simulink model "TSR_Scenario_001_cs"  (R2014b)
settings: Solver=ode5  SolverMode=SingleTasking  StartTime=0.0  StopTime=inf  FixedStep=1/100  RelTol=1e-3
PreLoadFcn:
  | mbxruntime.callbacks.PreLoadFcn(bdroot);
  | check_NUTS_defined;
  | 
  | assignin('base',['model_closed_' bdroot],false);
  | 
  | addpath('../includes_TSR/includes_TSR');
  | 
  | switch version('-release')
  | case {'2010a', '2010b', '2011a'}
  | addpath('../includes_TSR/ML2010b');
  | otherwise
  | addpath('../includes_TSR/ML2011b');
  | end
PostLoadFcn:
  | mbxruntime.callbacks.PostLoadFcn(bdroot);
InitFcn:
  | mbxruntime.callbacks.InitFcn(bdroot);
StartFcn:
  | mbxruntime.callbacks.StartFcn(bdroot);
StopFcn:
  | mbxruntime.callbacks.StopFcn(bdroot);
model workspace: external: MAT-File .\TSR_Scenario_001_cs_hws.mat (data not in the file)
undefined symbols (not defined in the file or in its folder): InitImageOutputDir, mbxruntime, OrientationPitch, OrientationRoll, PositionX, PositionY, PositionZ, tabledata, warningInitialVelocity, x0
undefined symbols (not defined in the file): SteeringColumn, SteeringWheel, TSR_Scenario_001_cs_0469e6db089af631, TSR_Scenario_001_cs_0511100212e7bc8e, TSR_Scenario_001_cs_0e7e9ae969427aac, TSR_Scenario_001_cs_1093386e49c2fe1f, TSR_Scenario_001_cs_112063adae8cf595, TSR_Scenario_001_cs_20f00d93cd5331c2, TSR_Scenario_001_cs_23e3512474fbfadc, TSR_Scenario_001_cs_366523e1554c6bf4, TSR_Scenario_001_cs_37bce4982c67337a, TSR_Scenario_001_cs_44e6164a5df50f45, TSR_Scenario_001_cs_4963ce12e7ff3247, TSR_Scenario_001_cs_4b3e01fa729ce73a, TSR_Scenario_001_cs_519c34727ce9f069, TSR_Scenario_001_cs_5b66ab60038399a1, TSR_Scenario_001_cs_5baa165dfa1afdcb, TSR_Scenario_001_cs_5f993ce39fa6372c, TSR_Scenario_001_cs_613fdf28e3ff7437, TSR_Scenario_001_cs_67b1406af835d622, TSR_Scenario_001_cs_6ad990c290286b94, TSR_Scenario_001_cs_6c412b69295984e1, TSR_Scenario_001_cs_6d4c0c06b1585ef3, TSR_Scenario_001_cs_6dd019d071bf1235, TSR_Scenario_001_cs_6e9f5883f1a78533, TSR_Scenario_001_cs_80f7223d9ac35404, TSR_Scenario_001_cs_8562b82d3c89ae57, TSR_Scenario_001_cs_8a3a0181ab0babfe, TSR_Scenario_001_cs_8c997348ce80deaf, TSR_Scenario_001_cs_925bd6a073d9fe25, TSR_Scenario_001_cs_961436216add6114, TSR_Scenario_001_cs_991a7959256b2c84, TSR_Scenario_001_cs_9a95ce2c2e753616, TSR_Scenario_001_cs_a98aa9562e8552a9, TSR_Scenario_001_cs_ab44ae81dbfb58cd, TSR_Scenario_001_cs_Actros_2541_2_Path_pathUniqueID, TSR_Scenario_001_cs_ae74836ade6bff5a, TSR_Scenario_001_cs_Audi_A8_1_Dynamics_Simple_initialPitch, TSR_Scenario_001_cs_Audi_A8_1_Dynamics_Simple_initialRoll, TSR_Scenario_001_cs_Audi_A8_1_Dynamics_Simple_initialX, TSR_Scenario_001_cs_Audi_A8_1_Dynamics_Simple_initialY, TSR_Scenario_001_cs_Audi_A8_1_Dynamics_Simple_initialYaw, TSR_Scenario_001_cs_Audi_A8_1_Dynamics_Simple_initialZ, TSR_Scenario_001_cs_Audi_A8_2_Path_pathUniqueID, TSR_Scenario_001_cs_Audi_A8_2_SpeedProfile_speedProfileUniqueID, TSR_Scenario_001_cs_b2eca4eb2fce349a, TSR_Scenario_001_cs_b7bac209c1f2549f, TSR_Scenario_001_cs_bf3dccb66d3255a4, TSR_Scenario_001_cs_bf4c1a5315e3f716, TSR_Scenario_001_cs_BMW_Z3_1_Path_pathUniqueID, TSR_Scenario_001_cs_BMW_Z3_1_SpeedProfile_speedProfileUniqueID, TSR_Scenario_001_cs_BMW_Z3_2_Path_pathUniqueID, TSR_Scenario_001_cs_BMW_Z3_2_SpeedProfile_speedProfileUniqueID, TSR_Scenario_001_cs_c4c8fc4bdece03a9, TSR_Scenario_001_cs_c964c86aa54ad92e, TSR_Scenario_001_cs_cb64d1ef85329755, TSR_Scenario_001_cs_Citroen_C3_1_Path_pathUniqueID, TSR_Scenario_001_cs_Citroen_C3_2_Path_pathUniqueID, TSR_Scenario_001_cs_Citroen_C3_3_Path_pathUniqueID, TSR_Scenario_001_cs_Citroen_C3_4_Path_pathUniqueID ... (+25)
libraries: simulink x21, PreScanSimulinkLibrary x17, simulink_extras x13
(part 1 of 30)
CloseFcn:
  | mbxruntime.callbacks.CloseFcn(bdroot);
  | evalin('base',['clear model_closed_' bdroot]);
settings Model: Creator=PRESCAN  LastModifiedBy=jenkins
settings DataIOCC: SignalLoggingSaveFormat=ModelDataLogs
settings OptimizationCC: InlineParams=on  ExpressionDepthLimit=2147483647  InitFltsAndDblsToZero=on
settings DebuggingCC: SaveWithParameterizedLinksMsg=none  UnderspecifiedInitializationDetection=Classic  MergeDetectMultiDrivingBlocksExec=none  SignalResolutionControl=TryResolveAllWithWarning  SolverPrmCheckMsg=none  MultiTaskDSMMsg=warning  MultiTaskCondExecSysMsg=none  FcnCallInpInsideContextMsg=UseLocalSettings  StateNameClashWarn=warning
settings ModelReferenceCC: UpdateModelReferenceTargets=IfOutOfDate
settings SFSimCC: SimParseCustomCode=off
settings SFSimCC: SimCustomHeaderCode=|
  | #include "prescan.h"
  | #include "prescan_platform.h"
settings RTWCC: IncludeERTFirstTime=on
settings GRTTargetCC: TargetFcnLib=ansi_tfl_tmw.mat  CombineOutputUpdateFcns=off  GRTInterface=on

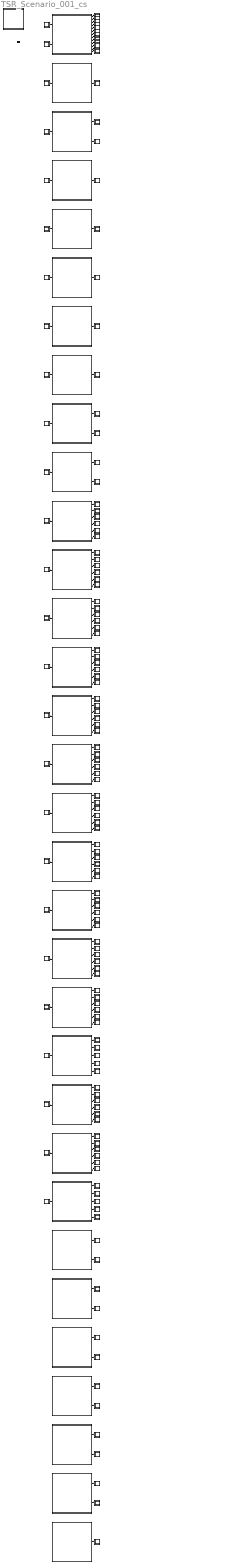
== system TSR_Scenario_001_cs ==
  note: Regenerate
  note: Simulink Mode
  note: Open Useful Blocks
  note: 2020.1.0
  note: Version:
  note: Author(s):
  note: N.A.
  note: Descriptive text:
  note: Demo Help
  note: ======
      | Num ID
      | ======
      | 1
      | 483
      | 484
      | 485
      | 828
      | 830
      | 486
      | 838
      | 959
      | 992
      | 999
      | 1001
      | 1002
      | 1003
      | 1004
      | 1005
      | 1006
      | 1007
      | 1008
      | 1009
      | 1010
      | 1011
      | 1012
      | 1000
  note: =============
      | OBU-Beacon ID
      | =============
  note: =======
      | Type ID
      | =======
      | 1
      | 3
      | 3
      | 7
      | 3
      | 7
      | 3
      | 1
      | 1
      | 1
      | 1
      | 1
      | 1
      | 1
      | 1
      | 1
      | 1
      | 1
      | 1
      | 1
      | 1
      | 1
      | 1
      | 3
  note: ========
      | Type Tag
      | ========
      | Car
      | Truck\Bus
      | Truck\Bus
      | Trailer
      | Truck\Bus
      | Trailer
      | Truck\Bus
      | Car
      | Car
      | Car
      | Car
      | Car
      | Car
      | Car
      | Car
      | Car
      | Car
      | Car
      | Car
      | Car
      | Car
      | Car
      | Car
      | Truck\Bus
  note: ==
      | SD
      | ==
      | Y
      | Y
      | Y
      | Y
      | Y
      | Y
      | Y
      | Y
      | Y
      | Y
      | Y
      | Y
      | Y
      | Y
      | Y
      | Y
      | Y
      | Y
      | Y
      | Y
      | Y
      | Y
      | Y
      | Y
  note: ==
      | CD
      | ==
      | N
      | N
      | N
      | N
      | N
      | N
      | N
      | N
      | N
      | N
      | N
      | N
      | N
      | N
      | N
      | N
      | N
      | N
      | N
      | N
      | N
      | N
      | N
      | N
  note: =======================
      | Name
      | =======================
      | Audi_A8_1
      | Nissan_Cabstar_1
      | Actros_1860_1
      | ContainerTrailer_DoubleAxle_1
      | Actros_1860_2
      | ContainerTrailer_DoubleAxle_2
      | Actros_2541_1
      | Toyota_Previa_1
      | Mazda_RX8_1
      | Mazda_RX8_2
      | Ford_Fiesta_1
      | BMW_Z3_1
      | Audi_A8_2
      | Citroen_C3_1
      | Citroen_C3_2
      | Toyota_Yaris_1
      | Fiat_Bravo_1
      | Citroen_C3_3
      | Toyota_Previa_2
      | Mazda_RX8_3
      | Fiat_Bravo_2
      | BMW_Z3_2
      | Citroen_C3_4
      | Actros_2541_2
  Actros_1860_1 : Subsystem  Tag=WorldObjectSubSystem  InitFcn=UniqueId = '1580';
      mask init:
      | modelPath = GenericModelHelper.getGenericModelFilePath('ModelDepo','Vehicles\Mercedes_Actros_1860\Mercedes_Actros_1860.pgmb','f4d262a59d21672e46677209b578f5e0');imagePath = GenericModelHelper.getCompilationPicture(modelPath, 'Mercedes_Actros_1860_HighPoly.png');
      mask Display: image(imread(imagePath));color('white');text(0, 0, ' ID=484\n')
  Actros_1860_2 : Subsystem  Tag=WorldObjectSubSystem  InitFcn=UniqueId = '1584';
      mask init: same as TSR_Scenario_001_cs/Actros_1860_1
      mask Display: image(imread(imagePath));color('white');text(0, 0, ' ID=828\n')
  Actros_2541_1 : Subsystem  Tag=WorldObjectSubSystem  InitFcn=UniqueId = '1588';
      mask init:
      | modelPath = GenericModelHelper.getGenericModelFilePath('ModelDepo','Vehicles\Mercedes_Actros_2541\Mercedes_Actros_2541.pgmb','2272788c542945e1b586df6742792b5a');imagePath = GenericModelHelper.getCompilationPicture(modelPath, 'Mercedes_Actros_2541_HighPoly.png');
      mask Display: image(imread(imagePath));color('white');text(0, 0, ' ID=486\n')
  Actros_2541_2 : Subsystem  Tag=WorldObjectSubSystem  InitFcn=UniqueId = '2575';
      mask init: same as TSR_Scenario_001_cs/Actros_2541_1
      mask Display: image(imread(imagePath));color('white');text(0, 0, ' ID=1000\n')
  Audi_A8_1 : Subsystem  Tag=WorldObjectSubSystem  InitFcn=UniqueId = '253';
      mask init:
      | modelPath = GenericModelHelper.getGenericModelFilePath('ModelDepo','Vehicles\Audi_A8\Audi_A8.pgmb','e33fe1ddcf3e8ae97caccbc8f2fa74ac');imagePath = GenericModelHelper.getCompilationPicture(modelPath, 'Audi_A8_HighPoly.png');
      mask Display: image(imread(imagePath));color('white');text(0, 0, ' ID=1\n')
  Audi_A8_1_Brake_light_left : Subsystem  Tag=actuator/BrakeLightL  Priority=0  LoadFcn=load('PreScanVisuLightActuatorData');load('PrescanRPYData');load('PrescanXYZData');load('PreScanRGBData')  mask(PreScan Sink Block: VisuActiveLight){}
      mask help:
      | The VisuActiveLight block provides a way for detailed animation of Light Sources, such as the indicator, brake, fog and main lights of a vehicle, or a light post.
      |
      | For more information, please click Help.
      settings: OpenFcn=open_system([gcb '/Actuator'],'mask')
      mask Help: eval('openHelp(209)')
      mask Display: image(imread('HeadLight.png'))
  Audi_A8_1_Brake_light_right : Subsystem  Tag=actuator/BrakeLightR  Priority=0  LoadFcn=load('PreScanVisuLightActuatorData');load('PrescanRPYData');load('PrescanXYZData');load('PreScanRGBData')  mask(PreScan Sink Block: VisuActiveLight){}
      mask help:
      | The VisuActiveLight block provides a way for detailed animation of Light Sources, such as the indicator, brake, fog and main lights of a vehicle, or a light post.
      |
      | For more information, please click Help.
      settings: OpenFcn=open_system([gcb '/Actuator'],'mask')
      mask Help: eval('openHelp(209)')
      mask Display: image(imread('HeadLight.png'))
  Audi_A8_1_Indicator_front_left : Subsystem  Tag=actuator/IndicatorFL  Priority=0  LoadFcn=load('PreScanVisuLightActuatorData');load('PrescanRPYData');load('PrescanXYZData');load('PreScanRGBData')  mask(PreScan Sink Block: VisuActiveLight){}
      mask help:
      | The VisuActiveLight block provides a way for detailed animation of Light Sources, such as the indicator, brake, fog and main lights of a vehicle, or a light post.
      |
      | For more information, please click Help.
      settings: OpenFcn=open_system([gcb '/Actuator'],'mask')
      mask Help: eval('openHelp(209)')
      mask Display: image(imread('HeadLight.png'))
  Audi_A8_1_Indicator_front_right : Subsystem  Tag=actuator/IndicatorFR  Priority=0  LoadFcn=load('PreScanVisuLightActuatorData');load('PrescanRPYData');load('PrescanXYZData');load('PreScanRGBData')  mask(PreScan Sink Block: VisuActiveLight){}
      mask help:
      | The VisuActiveLight block provides a way for detailed animation of Light Sources, such as the indicator, brake, fog and main lights of a vehicle, or a light post.
      |
      | For more information, please click Help.
      settings: OpenFcn=open_system([gcb '/Actuator'],'mask')
      mask Help: eval('openHelp(209)')
      mask Display: image(imread('HeadLight.png'))
  Audi_A8_1_Indicator_rear_left : Subsystem  Tag=actuator/IndicatorRL  Priority=0  LoadFcn=load('PreScanVisuLightActuatorData');load('PrescanRPYData');load('PrescanXYZData');load('PreScanRGBData')  mask(PreScan Sink Block: VisuActiveLight){}
      mask help:
      | The VisuActiveLight block provides a way for detailed animation of Light Sources, such as the indicator, brake, fog and main lights of a vehicle, or a light post.
      |
      | For more information, please click Help.
      settings: OpenFcn=open_system([gcb '/Actuator'],'mask')
      mask Help: eval('openHelp(209)')
      mask Display: image(imread('HeadLight.png'))
  Audi_A8_1_Indicator_rear_right : Subsystem  Tag=actuator/IndicatorRR  Priority=0  LoadFcn=load('PreScanVisuLightActuatorData');load('PrescanRPYData');load('PrescanXYZData');load('PreScanRGBData')  mask(PreScan Sink Block: VisuActiveLight){}
      mask help:
      | The VisuActiveLight block provides a way for detailed animation of Light Sources, such as the indicator, brake, fog and main lights of a vehicle, or a light post.
      |
      | For more information, please click Help.
      settings: OpenFcn=open_system([gcb '/Actuator'],'mask')
      mask Help: eval('openHelp(209)')
      mask Display: image(imread('HeadLight.png'))
  Audi_A8_2 : Subsystem  Tag=WorldObjectSubSystem  InitFcn=UniqueId = '1951';
      mask init: same as TSR_Scenario_001_cs/Audi_A8_1
      mask Display: image(imread(imagePath));color('white');text(0, 0, ' ID=1002\n')
  BMW_Z3_1 : Subsystem  Tag=WorldObjectSubSystem  InitFcn=UniqueId = '1948';
      mask init:
      | modelPath = GenericModelHelper.getGenericModelFilePath('ModelDepo','Vehicles\BMW_Z3\BMW_Z3.pgmb','9e6af5cc2d86218dad43975fd3a29d11');imagePath = GenericModelHelper.getCompilationPicture(modelPath, 'BMW_Z3_HighPoly.png');
      mask Display: image(imread(imagePath));color('white');text(0, 0, ' ID=1001\n')
  BMW_Z3_2 : Subsystem  Tag=WorldObjectSubSystem  InitFcn=UniqueId = '2024';
      mask init: same as TSR_Scenario_001_cs/BMW_Z3_1
      mask Display: image(imread(imagePath));color('white');text(0, 0, ' ID=1011\n')
  CameraSensor_1 : Subsystem  Tag=sensor/Camera/CameraSensor  Priority=30  mask(PreScan Source Block: Camera Sensor){}
      mask help: The Camera Sensor provides a color or monochrome image.
      settings: OpenFcn=open_system([gcb '/Sensor'],'mask')
      mask Help: eval('openHelp(457)')
      mask Display: image(imread('CameraSensor.png'))
  Citroen_C3_1 : Subsystem  Tag=WorldObjectSubSystem  InitFcn=UniqueId = '1955';
      mask init:
      | modelPath = GenericModelHelper.getGenericModelFilePath('ModelDepo','Vehicles\Citroen_C3\Citroen_C3.pgmb','e804ced06d50dbfc6a2202ab3ad01b0c');imagePath = GenericModelHelper.getCompilationPicture(modelPath, 'Citroen_C3_HighPoly.png');
      mask Display: image(imread(imagePath));color('white');text(0, 0, ' ID=1003\n')
  Citroen_C3_2 : Subsystem  Tag=WorldObjectSubSystem  InitFcn=UniqueId = '1958';
      mask init: same as TSR_Scenario_001_cs/Citroen_C3_1
      mask Display: image(imread(imagePath));color('white');text(0, 0, ' ID=1004\n')
  Citroen_C3_3 : Subsystem  Tag=WorldObjectSubSystem  InitFcn=UniqueId = '1967';
      mask init: same as TSR_Scenario_001_cs/Citroen_C3_1
      mask Display: image(imread(imagePath));color('white');text(0, 0, ' ID=1007\n')
  Citroen_C3_4 : Subsystem  Tag=WorldObjectSubSystem  InitFcn=UniqueId = '2027';
      mask init: same as TSR_Scenario_001_cs/Citroen_C3_1
      mask Display: image(imread(imagePath));color('white');text(0, 0, ' ID=1012\n')
  ContainerTrailer_DoubleAxle_1 : Subsystem  Tag=WorldObjectSubSystem  InitFcn=UniqueId = '1582';
      mask init:
      | modelPath = GenericModelHelper.getGenericModelFilePath('ModelDepo','Vehicles\Container\Container.pgmb','6d816eb34d08248d7edc89a1bf7f028c');imagePath = GenericModelHelper.getCompilationPicture(modelPath, 'Container_HighPoly.png');
      mask Display: image(imread(imagePath));color('white');text(0, 0, ' ID=485\n')
  ContainerTrailer_DoubleAxle_2 : Subsystem  Tag=WorldObjectSubSystem  InitFcn=UniqueId = '1586';
      mask init: same as TSR_Scenario_001_cs/ContainerTrailer_DoubleAxle_1
      mask Display: image(imread(imagePath));color('white');text(0, 0, ' ID=830\n')
  Controller : Subsystem  Description=8A3CD2955739A82C886C20AE3E253D78460D53180EE2C1B14CC08DF75A70BE77  Priority=-1  LoadFcn=load PreScanControllerData  mask(PreScan Simulation Controller){prescanversion='2020.1.0', ModelReferencing=off, TimeStep=1/100, ControlMode=0, PreScanExecutionMode=on, ControllerCount=0, ControllerIndex=0, ControllerOptions=''}
      mask prompts: prescanversion "PreScan Version"; ModelReferencing "Use Model Referencing"; TimeStep "Upload Period [s]"; ControlMode "Control Mode"; PreScanExecutionMode "Execution Mode"; ControllerCount "Controller Count"; ControllerIndex "Controller Index"; ControllerOptions "Controller Options"
      mask help:
      | Please do not remove this block from the compilation sheet,
      | as it connects the model to the PreScan environment.
      mask init:
      | model = bdroot(gcb);
      | ExperimentFile = mbxruntime.findExperimentFile(model,true); %relative path
      | 
      | [d1, d2, d3, prescandata] = prescan_Settings();
      | ModelDepo = fullfile(prescandata,'ModelDepo'); 
      | 
      | RTmode = mbxruntime.getRTMode(model);
      | 
      | SimulationMode = get_param(bdroot,'SimulationMode');
      | if strcmp(SimulationMode, 'rapid-accelerator')
      |     SimulationMode = 'external';
      | end
      | TargetName = get_param(bdroot,'SystemTargetFile');
      settings: ModelCloseFcn=assignin('base',['model_closed_' bdroot],true);
      mask Help: eval('openHelp(812)')
      mask Display: image(imread('prescanlogo.ico'))
  Fiat_Bravo_1 : Subsystem  Tag=WorldObjectSubSystem  InitFcn=UniqueId = '1964';
      mask init:
      | modelPath = GenericModelHelper.getGenericModelFilePath('ModelDepo','Vehicles\Fiat_Bravo\Fiat_Bravo.pgmb','a97eb0ec4093646e5d079d2ab9a2eab7');imagePath = GenericModelHelper.getCompilationPicture(modelPath, 'Fiat_Bravo_HighPoly.png');
      mask Display: image(imread(imagePath));color('white');text(0, 0, ' ID=1006\n')
  Fiat_Bravo_2 : Subsystem  Tag=WorldObjectSubSystem  InitFcn=UniqueId = '2021';
      mask init: same as TSR_Scenario_001_cs/Fiat_Bravo_1
      mask Display: image(imread(imagePath));color('white');text(0, 0, ' ID=1010\n')
  Ford_Fiesta_1 : Subsystem  Tag=WorldObjectSubSystem  InitFcn=UniqueId = '1934';
      mask init:
      | modelPath = GenericModelHelper.getGenericModelFilePath('ModelDepo','Vehicles\Ford_Fiesta\Ford_Fiesta.pgmb','fe2c7a73e0a60cba76689b71cd1bb76a');imagePath = GenericModelHelper.getCompilationPicture(modelPath, 'Ford_Fiesta_HighPoly.png');
      mask Display: image(imread(imagePath));color('white');text(0, 0, ' ID=999\n')
  HighwayOverhang_1 : Subsystem  Tag=WorldObjectSubSystem  InitFcn=UniqueId = '1876';
      mask init:
      | imagePath=which('HighwayOverhang.jpg');
      mask Display: image(imread(imagePath));color('white');text(0, 0, ' ID=115\n')
  HighwayOverhang_2 : Subsystem  Tag=WorldObjectSubSystem  InitFcn=UniqueId = '1877';
      mask init:
      | imagePath=which('HighwayOverhang.jpg');
      mask Display: image(imread(imagePath));color('white');text(0, 0, ' ID=973\n')
  HighwayOverhang_3 : Subsystem  Tag=WorldObjectSubSystem  InitFcn=UniqueId = '1890';
      mask init:
      | imagePath=which('HighwayOverhang.jpg');
      mask Display: image(imread(imagePath));color('white');text(0, 0, ' ID=985\n')
  HighwayOverhang_4 : Subsystem  Tag=WorldObjectSubSystem  InitFcn=UniqueId = '1898';
      mask init:
      | imagePath=which('HighwayOverhang.jpg');
      mask Display: image(imread(imagePath));color('white');text(0, 0, ' ID=988\n')
  HighwayOverhang_5 : Subsystem  Tag=WorldObjectSubSystem  InitFcn=UniqueId = '1909';
      mask init:
      | imagePath=which('HighwayOverhang.jpg');
      mask Display: image(imread(imagePath));color('white');text(0, 0, ' ID=993\n')
  HighwayOverhang_6 : Subsystem  Tag=WorldObjectSubSystem  InitFcn=UniqueId = '1914';
      mask init:
      | imagePath=which('HighwayOverhang.jpg');
      mask Display: image(imread(imagePath));color('white');text(0, 0, ' ID=994\n')
  HighwayOverhang_7 : Subsystem  Tag=WorldObjectSubSystem  InitFcn=UniqueId = '2612';
      mask init:
      | imagePath=which('HighwayOverhang.jpg');
      mask Display: image(imread(imagePath));color('white');text(0, 0, ' ID=1505\n')
  Mazda_RX8_1 : Subsystem  Tag=WorldObjectSubSystem  InitFcn=UniqueId = '1863';
      mask init:
      | modelPath = GenericModelHelper.getGenericModelFilePath('ModelDepo','Vehicles\Mazda_RX8\Mazda_RX8.pgmb','1e55a2e40efa576b7f4fb93bae35d605');imagePath = GenericModelHelper.getCompilationPicture(modelPath, 'Mazda_RX8_HighPoly.png');
      mask Display: image(imread(imagePath));color('white');text(0, 0, ' ID=959\n')
  Mazda_RX8_2 : Subsystem  Tag=WorldObjectSubSystem  InitFcn=UniqueId = '1929';
      mask init: same as TSR_Scenario_001_cs/Mazda_RX8_1
      mask Display: image(imread(imagePath));color('white');text(0, 0, ' ID=992\n')
  Mazda_RX8_3 : Subsystem  Tag=WorldObjectSubSystem  InitFcn=UniqueId = '1973';
      mask init: same as TSR_Scenario_001_cs/Mazda_RX8_1
      mask Display: image(imread(imagePath));color('white');text(0, 0, ' ID=1009\n')
  Nissan_Cabstar_1 : Subsystem  Tag=WorldObjectSubSystem  InitFcn=UniqueId = '1579';
      mask init:
      | modelPath = GenericModelHelper.getGenericModelFilePath('ModelDepo','Vehicles\Nissan_Cabstar\Nissan_Cabstar.pgmb','dd076fdae311093c5436e82e6c23dc23');imagePath = GenericModelHelper.getCompilationPicture(modelPath, 'Nissan_Cabstar_HighPoly.png');
      mask Display: image(imread(imagePath));color('white');text(0, 0, ' ID=483\n')
  PreScanTerminator : Subsystem  Tag=PreScanTerminator  Priority=999  LoadFcn=load PrescanTerminatorData  mask(PreScan Simulation Terminator){TimeStep=1/100}
      mask prompts: TimeStep "Upload Period [s]"
      mask help:
      | Please do not remove this block from the compilation sheet as it
      | connects the model to the PreScan environment.
      mask Help: eval('openHelp(812)')
      mask Display: image(imread('prescanlogo.ico'))
  SELF_Actros_1860_1 : Subsystem  Tag=sensor/SelfPort  Priority=30  LoadFcn=load('PreScanSelfSensorData.mat')  mask(PreScan Source Block: SELF){}
      mask help:
      | The SELF port shows (state) information of the actor itself. The outputs are position in the experiment's axis system and the GPS coordinates, and the object's absolute velocity and compass heading.
      |
      | For more information, please click Help.
      settings: OpenFcn=open_system([gcb '/Sensor'],'mask')
      mask Help: eval('openHelp(462)')
      mask Display: image(imread('GPS.png'))
  SELF_Actros_1860_2 : Subsystem  Tag=sensor/SelfPort  Priority=30  LoadFcn=load('PreScanSelfSensorData.mat')  mask(PreScan Source Block: SELF){}
      mask help:
      | The SELF port shows (state) information of the actor itself. The outputs are position in the experiment's axis system and the GPS coordinates, and the object's absolute velocity and compass heading.
      |
      | For more information, please click Help.
      settings: OpenFcn=open_system([gcb '/Sensor'],'mask')
      mask Help: eval('openHelp(462)')
      mask Display: image(imread('GPS.png'))
  SELF_Actros_2541_1 : Subsystem  Tag=sensor/SelfPort  Priority=30  LoadFcn=load('PreScanSelfSensorData.mat')  mask(PreScan Source Block: SELF){}
      mask help:
      | The SELF port shows (state) information of the actor itself. The outputs are position in the experiment's axis system and the GPS coordinates, and the object's absolute velocity and compass heading.
      |
      | For more information, please click Help.
      settings: OpenFcn=open_system([gcb '/Sensor'],'mask')
      mask Help: eval('openHelp(462)')
      mask Display: image(imread('GPS.png'))
  SELF_Actros_2541_2 : Subsystem  Tag=sensor/SelfPort  Priority=30  LoadFcn=load('PreScanSelfSensorData.mat')  mask(PreScan Source Block: SELF){}
      mask help:
      | The SELF port shows (state) information of the actor itself. The outputs are position in the experiment's axis system and the GPS coordinates, and the object's absolute velocity and compass heading.
      |
      | For more information, please click Help.
      settings: OpenFcn=open_system([gcb '/Sensor'],'mask')
      mask Help: eval('openHelp(462)')
      mask Display: image(imread('GPS.png'))
  SELF_Audi_A8_1 : Subsystem  Tag=sensor/SelfPort  Priority=30  LoadFcn=load('PreScanSelfSensorData.mat')  mask(PreScan Source Block: SELF){}
      mask help:
      | The SELF port shows (state) information of the actor itself. The outputs are position in the experiment's axis system and the GPS coordinates, and the object's absolute velocity and compass heading.
      |
      | For more information, please click Help.
      settings: OpenFcn=open_system([gcb '/Sensor'],'mask')
      mask Help: eval('openHelp(462)')
      mask Display: image(imread('GPS.png'))
  SELF_Audi_A8_2 : Subsystem  Tag=sensor/SelfPort  Priority=30  LoadFcn=load('PreScanSelfSensorData.mat')  mask(PreScan Source Block: SELF){}
      mask help:
      | The SELF port shows (state) information of the actor itself. The outputs are position in the experiment's axis system and the GPS coordinates, and the object's absolute velocity and compass heading.
      |
      | For more information, please click Help.
      settings: OpenFcn=open_system([gcb '/Sensor'],'mask')
      mask Help: eval('openHelp(462)')
      mask Display: image(imread('GPS.png'))
  SELF_BMW_Z3_1 : Subsystem  Tag=sensor/SelfPort  Priority=30  LoadFcn=load('PreScanSelfSensorData.mat')  mask(PreScan Source Block: SELF){}
      mask help:
      | The SELF port shows (state) information of the actor itself. The outputs are position in the experiment's axis system and the GPS coordinates, and the object's absolute velocity and compass heading.
      |
      | For more information, please click Help.
      settings: OpenFcn=open_system([gcb '/Sensor'],'mask')
      mask Help: eval('openHelp(462)')
      mask Display: image(imread('GPS.png'))
  SELF_BMW_Z3_2 : Subsystem  Tag=sensor/SelfPort  Priority=30  LoadFcn=load('PreScanSelfSensorData.mat')  mask(PreScan Source Block: SELF){}
      mask help:
      | The SELF port shows (state) information of the actor itself. The outputs are position in the experiment's axis system and the GPS coordinates, and the object's absolute velocity and compass heading.
      |
      | For more information, please click Help.
      settings: OpenFcn=open_system([gcb '/Sensor'],'mask')
      mask Help: eval('openHelp(462)')
      mask Display: image(imread('GPS.png'))
  SELF_Citroen_C3_1 : Subsystem  Tag=sensor/SelfPort  Priority=30  LoadFcn=load('PreScanSelfSensorData.mat')  mask(PreScan Source Block: SELF){}
      mask help:
      | The SELF port shows (state) information of the actor itself. The outputs are position in the experiment's axis system and the GPS coordinates, and the object's absolute velocity and compass heading.
      |
      | For more information, please click Help.
      settings: OpenFcn=open_system([gcb '/Sensor'],'mask')
      mask Help: eval('openHelp(462)')
      mask Display: image(imread('GPS.png'))
  SELF_Citroen_C3_2 : Subsystem  Tag=sensor/SelfPort  Priority=30  LoadFcn=load('PreScanSelfSensorData.mat')  mask(PreScan Source Block: SELF){}
      mask help:
      | The SELF port shows (state) information of the actor itself. The outputs are position in the experiment's axis system and the GPS coordinates, and the object's absolute velocity and compass heading.
      |
      | For more information, please click Help.
      settings: OpenFcn=open_system([gcb '/Sensor'],'mask')
      mask Help: eval('openHelp(462)')
      mask Display: image(imread('GPS.png'))
  SELF_Citroen_C3_3 : Subsystem  Tag=sensor/SelfPort  Priority=30  LoadFcn=load('PreScanSelfSensorData.mat')  mask(PreScan Source Block: SELF){}
      mask help:
      | The SELF port shows (state) information of the actor itself. The outputs are position in the experiment's axis system and the GPS coordinates, and the object's absolute velocity and compass heading.
      |
      | For more information, please click Help.
      settings: OpenFcn=open_system([gcb '/Sensor'],'mask')
      mask Help: eval('openHelp(462)')
      mask Display: image(imread('GPS.png'))
  SELF_Citroen_C3_4 : Subsystem  Tag=sensor/SelfPort  Priority=30  LoadFcn=load('PreScanSelfSensorData.mat')  mask(PreScan Source Block: SELF){}
      mask help:
      | The SELF port shows (state) information of the actor itself. The outputs are position in the experiment's axis system and the GPS coordinates, and the object's absolute velocity and compass heading.
      |
      | For more information, please click Help.
      settings: OpenFcn=open_system([gcb '/Sensor'],'mask')
      mask Help: eval('openHelp(462)')
      mask Display: image(imread('GPS.png'))
  SELF_ContainerTrailer_DoubleAxle_1 : Subsystem  Tag=sensor/SelfPort  Priority=30  LoadFcn=load('PreScanSelfSensorData.mat')  mask(PreScan Source Block: SELF){}
      mask help:
      | The SELF port shows (state) information of the actor itself. The outputs are position in the experiment's axis system and the GPS coordinates, and the object's absolute velocity and compass heading.
      |
      | For more information, please click Help.
      settings: OpenFcn=open_system([gcb '/Sensor'],'mask')
      mask Help: eval('openHelp(462)')
      mask Display: image(imread('GPS.png'))
  SELF_ContainerTrailer_DoubleAxle_2 : Subsystem  Tag=sensor/SelfPort  Priority=30  LoadFcn=load('PreScanSelfSensorData.mat')  mask(PreScan Source Block: SELF){}
      mask help:
      | The SELF port shows (state) information of the actor itself. The outputs are position in the experiment's axis system and the GPS coordinates, and the object's absolute velocity and compass heading.
      |
      | For more information, please click Help.
      settings: OpenFcn=open_system([gcb '/Sensor'],'mask')
      mask Help: eval('openHelp(462)')
      mask Display: image(imread('GPS.png'))
  SELF_Fiat_Bravo_1 : Subsystem  Tag=sensor/SelfPort  Priority=30  LoadFcn=load('PreScanSelfSensorData.mat')  mask(PreScan Source Block: SELF){}
      mask help:
      | The SELF port shows (state) information of the actor itself. The outputs are position in the experiment's axis system and the GPS coordinates, and the object's absolute velocity and compass heading.
      |
      | For more information, please click Help.
      settings: OpenFcn=open_system([gcb '/Sensor'],'mask')
      mask Help: eval('openHelp(462)')
      mask Display: image(imread('GPS.png'))
  SELF_Fiat_Bravo_2 : Subsystem  Tag=sensor/SelfPort  Priority=30  LoadFcn=load('PreScanSelfSensorData.mat')  mask(PreScan Source Block: SELF){}
      mask help:
      | The SELF port shows (state) information of the actor itself. The outputs are position in the experiment's axis system and the GPS coordinates, and the object's absolute velocity and compass heading.
      |
      | For more information, please click Help.
      settings: OpenFcn=open_system([gcb '/Sensor'],'mask')
      mask Help: eval('openHelp(462)')
      mask Display: image(imread('GPS.png'))
  SELF_Ford_Fiesta_1 : Subsystem  Tag=sensor/SelfPort  Priority=30  LoadFcn=load('PreScanSelfSensorData.mat')  mask(PreScan Source Block: SELF){}
      mask help:
      | The SELF port shows (state) information of the actor itself. The outputs are position in the experiment's axis system and the GPS coordinates, and the object's absolute velocity and compass heading.
      |
      | For more information, please click Help.
      settings: OpenFcn=open_system([gcb '/Sensor'],'mask')
      mask Help: eval('openHelp(462)')
      mask Display: image(imread('GPS.png'))
  SELF_Mazda_RX8_1 : Subsystem  Tag=sensor/SelfPort  Priority=30  LoadFcn=load('PreScanSelfSensorData.mat')  mask(PreScan Source Block: SELF){}
      mask help:
      | The SELF port shows (state) information of the actor itself. The outputs are position in the experiment's axis system and the GPS coordinates, and the object's absolute velocity and compass heading.
      |
      | For more information, please click Help.
      settings: OpenFcn=open_system([gcb '/Sensor'],'mask')
      mask Help: eval('openHelp(462)')
      mask Display: image(imread('GPS.png'))
  SELF_Mazda_RX8_2 : Subsystem  Tag=sensor/SelfPort  Priority=30  LoadFcn=load('PreScanSelfSensorData.mat')  mask(PreScan Source Block: SELF){}
      mask help:
      | The SELF port shows (state) information of the actor itself. The outputs are position in the experiment's axis system and the GPS coordinates, and the object's absolute velocity and compass heading.
      |
      | For more information, please click Help.
      settings: OpenFcn=open_system([gcb '/Sensor'],'mask')
      mask Help: eval('openHelp(462)')
      mask Display: image(imread('GPS.png'))
  SELF_Mazda_RX8_3 : Subsystem  Tag=sensor/SelfPort  Priority=30  LoadFcn=load('PreScanSelfSensorData.mat')  mask(PreScan Source Block: SELF){}
      mask help:
      | The SELF port shows (state) information of the actor itself. The outputs are position in the experiment's axis system and the GPS coordinates, and the object's absolute velocity and compass heading.
      |
      | For more information, please click Help.
      settings: OpenFcn=open_system([gcb '/Sensor'],'mask')
      mask Help: eval('openHelp(462)')
      mask Display: image(imread('GPS.png'))
  SELF_Nissan_Cabstar_1 : Subsystem  Tag=sensor/SelfPort  Priority=30  LoadFcn=load('PreScanSelfSensorData.mat')  mask(PreScan Source Block: SELF){}
      mask help:
      | The SELF port shows (state) information of the actor itself. The outputs are position in the experiment's axis system and the GPS coordinates, and the object's absolute velocity and compass heading.
      |
      | For more information, please click Help.
      settings: OpenFcn=open_system([gcb '/Sensor'],'mask')
      mask Help: eval('openHelp(462)')
      mask Display: image(imread('GPS.png'))
  SELF_Sphere_1 : Subsystem  Tag=sensor/SelfPort  Priority=30  LoadFcn=load('PreScanSelfSensorData.mat')  mask(PreScan Source Block: SELF){}
      mask help:
      | The SELF port shows (state) information of the actor itself. The outputs are position in the experiment's axis system and the GPS coordinates, and the object's absolute velocity and compass heading.
      |
      | For more information, please click Help.
      settings: OpenFcn=open_system([gcb '/Sensor'],'mask')
      mask Help: eval('openHelp(462)')
      mask Display: image(imread('GPS.png'))
  SELF_Toyota_Previa_1 : Subsystem  Tag=sensor/SelfPort  Priority=30  LoadFcn=load('PreScanSelfSensorData.mat')  mask(PreScan Source Block: SELF){}
      mask help:
      | The SELF port shows (state) information of the actor itself. The outputs are position in the experiment's axis system and the GPS coordinates, and the object's absolute velocity and compass heading.
      |
      | For more information, please click Help.
      settings: OpenFcn=open_system([gcb '/Sensor'],'mask')
      mask Help: eval('openHelp(462)')
      mask Display: image(imread('GPS.png'))
  SELF_Toyota_Previa_2 : Subsystem  Tag=sensor/SelfPort  Priority=30  LoadFcn=load('PreScanSelfSensorData.mat')  mask(PreScan Source Block: SELF){}
      mask help:
      | The SELF port shows (state) information of the actor itself. The outputs are position in the experiment's axis system and the GPS coordinates, and the object's absolute velocity and compass heading.
      |
      | For more information, please click Help.
      settings: OpenFcn=open_system([gcb '/Sensor'],'mask')
      mask Help: eval('openHelp(462)')
      mask Display: image(imread('GPS.png'))
  SELF_Toyota_Yaris_1 : Subsystem  Tag=sensor/SelfPort  Priority=30  LoadFcn=load('PreScanSelfSensorData.mat')  mask(PreScan Source Block: SELF){}
      mask help:
      | The SELF port shows (state) information of the actor itself. The outputs are position in the experiment's axis system and the GPS coordinates, and the object's absolute velocity and compass heading.
      |
      | For more information, please click Help.
      settings: OpenFcn=open_system([gcb '/Sensor'],'mask')
      mask Help: eval('openHelp(462)')
      mask Display: image(imread('GPS.png'))
  STATE_Actros_1860_1_bus : Subsystem  Tag=actuator/StatePort  Priority=0  LoadFcn=load('PreScanStateActuatorData.mat')  mask(PreScan Sink Block: State){}
      mask help:
      | The Actor State contains a vector signal of size (9x1), containing the following signals:
      |
      | -  Position    	(x,y,z)             	[m]
      | -  Velocity    	(vx,vy,vz)         	[m/s]
      | -  Angles       	(Roll, Pitch, Yaw)	[rad]
      |
      | The Actor state is defined in the global axis system.
      | The state is superponed on the Initial position defined in the GUI.
      |
      | For more information, please click Help.
      settings: OpenFcn=open_system([gcb '/Actuator'],'mask')
      mask Help: eval('openHelp(222)')
      mask Display: image(imread('State.png'))
  STATE_Actros_1860_2_bus : Subsystem  Tag=actuator/StatePort  Priority=0  LoadFcn=load('PreScanStateActuatorData.mat')  mask(PreScan Sink Block: State){}
      mask help:
      | The Actor State contains a vector signal of size (9x1), containing the following signals:
      |
      | -  Position    	(x,y,z)             	[m]
      | -  Velocity    	(vx,vy,vz)         	[m/s]
      | -  Angles       	(Roll, Pitch, Yaw)	[rad]
      |
      | The Actor state is defined in the global axis system.
      | The state is superponed on the Initial position defined in the GUI.
      |
      | For more information, please click Help.
      settings: OpenFcn=open_system([gcb '/Actuator'],'mask')
      mask Help: eval('openHelp(222)')
      mask Display: image(imread('State.png'))
  STATE_Actros_2541_1_bus : Subsystem  Tag=actuator/StatePort  Priority=0  LoadFcn=load('PreScanStateActuatorData.mat')  mask(PreScan Sink Block: State){}
      mask help:
      | The Actor State contains a vector signal of size (9x1), containing the following signals:
      |
      | -  Position    	(x,y,z)             	[m]
      | -  Velocity    	(vx,vy,vz)         	[m/s]
      | -  Angles       	(Roll, Pitch, Yaw)	[rad]
      |
      | The Actor state is defined in the global axis system.
      | The state is superponed on the Initial position defined in the GUI.
      |
      | For more information, please click Help.
      settings: OpenFcn=open_system([gcb '/Actuator'],'mask')
      mask Help: eval('openHelp(222)')
      mask Display: image(imread('State.png'))
  STATE_Actros_2541_2_bus : Subsystem  Tag=actuator/StatePort  Priority=0  LoadFcn=load('PreScanStateActuatorData.mat')  mask(PreScan Sink Block: State){}
      mask help:
      | The Actor State contains a vector signal of size (9x1), containing the following signals:
      |
      | -  Position    	(x,y,z)             	[m]
      | -  Velocity    	(vx,vy,vz)         	[m/s]
      | -  Angles       	(Roll, Pitch, Yaw)	[rad]
      |
      | The Actor state is defined in the global axis system.
      | The state is superponed on the Initial position defined in the GUI.
      |
      | For more information, please click Help.
      settings: OpenFcn=open_system([gcb '/Actuator'],'mask')
      mask Help: eval('openHelp(222)')
      mask Display: image(imread('State.png'))
  STATE_Audi_A8_1_bus : Subsystem  Tag=actuator/StatePort  Priority=0  LoadFcn=load('PreScanStateActuatorData.mat')  mask(PreScan Sink Block: State){}
      mask help:
      | The Actor State contains a vector signal of size (9x1), containing the following signals:
      |
      | -  Position    	(x,y,z)             	[m]
      | -  Velocity    	(vx,vy,vz)         	[m/s]
      | -  Angles       	(Roll, Pitch, Yaw)	[rad]
      |
      | The Actor state is defined in the global axis system.
      | The state is superponed on the Initial position defined in the GUI.
      |
      | For more information, please click Help.
      settings: OpenFcn=open_system([gcb '/Actuator'],'mask')
      mask Help: eval('openHelp(222)')
      mask Display: image(imread('State.png'))
  STATE_Audi_A8_2_bus : Subsystem  Tag=actuator/StatePort  Priority=0  LoadFcn=load('PreScanStateActuatorData.mat')  mask(PreScan Sink Block: State){}
      mask help:
      | The Actor State contains a vector signal of size (9x1), containing the following signals:
      |
      | -  Position    	(x,y,z)             	[m]
      | -  Velocity    	(vx,vy,vz)         	[m/s]
      | -  Angles       	(Roll, Pitch, Yaw)	[rad]
      |
      | The Actor state is defined in the global axis system.
      | The state is superponed on the Initial position defined in the GUI.
      |
      | For more information, please click Help.
      settings: OpenFcn=open_system([gcb '/Actuator'],'mask')
      mask Help: eval('openHelp(222)')
      mask Display: image(imread('State.png'))
  STATE_BMW_Z3_1_bus : Subsystem  Tag=actuator/StatePort  Priority=0  LoadFcn=load('PreScanStateActuatorData.mat')  mask(PreScan Sink Block: State){}
      mask help:
      | The Actor State contains a vector signal of size (9x1), containing the following signals:
      |
      | -  Position    	(x,y,z)             	[m]
      | -  Velocity    	(vx,vy,vz)         	[m/s]
      | -  Angles       	(Roll, Pitch, Yaw)	[rad]
      |
      | The Actor state is defined in the global axis system.
      | The state is superponed on the Initial position defined in the GUI.
      |
      | For more information, please click Help.
      settings: OpenFcn=open_system([gcb '/Actuator'],'mask')
      mask Help: eval('openHelp(222)')
      mask Display: image(imread('State.png'))
  STATE_BMW_Z3_2_bus : Subsystem  Tag=actuator/StatePort  Priority=0  LoadFcn=load('PreScanStateActuatorData.mat')  mask(PreScan Sink Block: State){}
      mask help:
      | The Actor State contains a vector signal of size (9x1), containing the following signals:
      |
      | -  Position    	(x,y,z)             	[m]
      | -  Velocity    	(vx,vy,vz)         	[m/s]
      | -  Angles       	(Roll, Pitch, Yaw)	[rad]
      |
      | The Actor state is defined in the global axis system.
      | The state is superponed on the Initial position defined in the GUI.
      |
      | For more information, please click Help.
      settings: OpenFcn=open_system([gcb '/Actuator'],'mask')
      mask Help: eval('openHelp(222)')
      mask Display: image(imread('State.png'))
  STATE_Citroen_C3_1_bus : Subsystem  Tag=actuator/StatePort  Priority=0  LoadFcn=load('PreScanStateActuatorData.mat')  mask(PreScan Sink Block: State){}
      mask help:
      | The Actor State contains a vector signal of size (9x1), containing the following signals:
      |
      | -  Position    	(x,y,z)             	[m]
      | -  Velocity    	(vx,vy,vz)         	[m/s]
      | -  Angles       	(Roll, Pitch, Yaw)	[rad]
      |
      | The Actor state is defined in the global axis system.
      | The state is superponed on the Initial position defined in the GUI.
      |
      | For more information, please click Help.
      settings: OpenFcn=open_system([gcb '/Actuator'],'mask')
      mask Help: eval('openHelp(222)')
      mask Display: image(imread('State.png'))
  STATE_Citroen_C3_2_bus : Subsystem  Tag=actuator/StatePort  Priority=0  LoadFcn=load('PreScanStateActuatorData.mat')  mask(PreScan Sink Block: State){}
      mask help:
      | The Actor State contains a vector signal of size (9x1), containing the following signals:
      |
      | -  Position    	(x,y,z)             	[m]
      | -  Velocity    	(vx,vy,vz)         	[m/s]
      | -  Angles       	(Roll, Pitch, Yaw)	[rad]
      |
      | The Actor state is defined in the global axis system.
      | The state is superponed on the Initial position defined in the GUI.
      |
      | For more information, please click Help.
      settings: OpenFcn=open_system([gcb '/Actuator'],'mask')
      mask Help: eval('openHelp(222)')
      mask Display: image(imread('State.png'))
  STATE_Citroen_C3_3_bus : Subsystem  Tag=actuator/StatePort  Priority=0  LoadFcn=load('PreScanStateActuatorData.mat')  mask(PreScan Sink Block: State){}
      mask help:
      | The Actor State contains a vector signal of size (9x1), containing the following signals:
      |
      | -  Position    	(x,y,z)             	[m]
      | -  Velocity    	(vx,vy,vz)         	[m/s]
      | -  Angles       	(Roll, Pitch, Yaw)	[rad]
      |
      | The Actor state is defined in the global axis system.
      | The state is superponed on the Initial position defined in the GUI.
      |
      | For more information, please click Help.
      settings: OpenFcn=open_system([gcb '/Actuator'],'mask')
      mask Help: eval('openHelp(222)')
      mask Display: image(imread('State.png'))
  STATE_Citroen_C3_4_bus : Subsystem  Tag=actuator/StatePort  Priority=0  LoadFcn=load('PreScanStateActuatorData.mat')  mask(PreScan Sink Block: State){}
      mask help:
      | The Actor State contains a vector signal of size (9x1), containing the following signals:
      |
      | -  Position    	(x,y,z)             	[m]
      | -  Velocity    	(vx,vy,vz)         	[m/s]
      | -  Angles       	(Roll, Pitch, Yaw)	[rad]
      |
      | The Actor state is defined in the global axis system.
      | The state is superponed on the Initial position defined in the GUI.
      |
      | For more information, please click Help.
      settings: OpenFcn=open_system([gcb '/Actuator'],'mask')
      mask Help: eval('openHelp(222)')
      mask Display: image(imread('State.png'))
  STATE_ContainerTrailer_DoubleAxle_1_bus : Subsystem  Tag=actuator/StatePort  Priority=0  LoadFcn=load('PreScanStateActuatorData.mat')  mask(PreScan Sink Block: State){}
      mask help:
      | The Actor State contains a vector signal of size (9x1), containing the following signals:
      |
      | -  Position    	(x,y,z)             	[m]
      | -  Velocity    	(vx,vy,vz)         	[m/s]
      | -  Angles       	(Roll, Pitch, Yaw)	[rad]
      |
      | The Actor state is defined in the global axis system.
      | The state is superponed on the Initial position defined in the GUI.
      |
      | For more information, please click Help.
      settings: OpenFcn=open_system([gcb '/Actuator'],'mask')
      mask Help: eval('openHelp(222)')
      mask Display: image(imread('State.png'))
  STATE_ContainerTrailer_DoubleAxle_2_bus : Subsystem  Tag=actuator/StatePort  Priority=0  LoadFcn=load('PreScanStateActuatorData.mat')  mask(PreScan Sink Block: State){}
      mask help:
      | The Actor State contains a vector signal of size (9x1), containing the following signals:
      |
      | -  Position    	(x,y,z)             	[m]
      | -  Velocity    	(vx,vy,vz)         	[m/s]
      | -  Angles       	(Roll, Pitch, Yaw)	[rad]
      |
      | The Actor state is defined in the global axis system.
      | The state is superponed on the Initial position defined in the GUI.
      |
      | For more information, please click Help.
      settings: OpenFcn=open_system([gcb '/Actuator'],'mask')
      mask Help: eval('openHelp(222)')
      mask Display: image(imread('State.png'))
  STATE_Fiat_Bravo_1_bus : Subsystem  Tag=actuator/StatePort  Priority=0  LoadFcn=load('PreScanStateActuatorData.mat')  mask(PreScan Sink Block: State){}
      mask help:
      | The Actor State contains a vector signal of size (9x1), containing the following signals:
      |
      | -  Position    	(x,y,z)             	[m]
      | -  Velocity    	(vx,vy,vz)         	[m/s]
      | -  Angles       	(Roll, Pitch, Yaw)	[rad]
      |
      | The Actor state is defined in the global axis system.
      | The state is superponed on the Initial position defined in the GUI.
      |
      | For more information, please click Help.
      settings: OpenFcn=open_system([gcb '/Actuator'],'mask')
      mask Help: eval('openHelp(222)')
      mask Display: image(imread('State.png'))
  STATE_Fiat_Bravo_2_bus : Subsystem  Tag=actuator/StatePort  Priority=0  LoadFcn=load('PreScanStateActuatorData.mat')  mask(PreScan Sink Block: State){}
      mask help:
      | The Actor State contains a vector signal of size (9x1), containing the following signals:
      |
      | -  Position    	(x,y,z)             	[m]
      | -  Velocity    	(vx,vy,vz)         	[m/s]
      | -  Angles       	(Roll, Pitch, Yaw)	[rad]
      |
      | The Actor state is defined in the global axis system.
      | The state is superponed on the Initial position defined in the GUI.
      |
      | For more information, please click Help.
      settings: OpenFcn=open_system([gcb '/Actuator'],'mask')
      mask Help: eval('openHelp(222)')
      mask Display: image(imread('State.png'))
  STATE_Ford_Fiesta_1_bus : Subsystem  Tag=actuator/StatePort  Priority=0  LoadFcn=load('PreScanStateActuatorData.mat')  mask(PreScan Sink Block: State){}
      mask help:
      | The Actor State contains a vector signal of size (9x1), containing the following signals:
      |
      | -  Position    	(x,y,z)             	[m]
      | -  Velocity    	(vx,vy,vz)         	[m/s]
      | -  Angles       	(Roll, Pitch, Yaw)	[rad]
      |
      | The Actor state is defined in the global axis system.
      | The state is superponed on the Initial position defined in the GUI.
      |
      | For more information, please click Help.
      settings: OpenFcn=open_system([gcb '/Actuator'],'mask')
      mask Help: eval('openHelp(222)')
      mask Display: image(imread('State.png'))
  STATE_Mazda_RX8_1_bus : Subsystem  Tag=actuator/StatePort  Priority=0  LoadFcn=load('PreScanStateActuatorData.mat')  mask(PreScan Sink Block: State){}
      mask help:
      | The Actor State contains a vector signal of size (9x1), containing the following signals:
      |
      | -  Position    	(x,y,z)             	[m]
      | -  Velocity    	(vx,vy,vz)         	[m/s]
      | -  Angles       	(Roll, Pitch, Yaw)	[rad]
      |
      | The Actor state is defined in the global axis system.
      | The state is superponed on the Initial position defined in the GUI.
      |
      | For more information, please click Help.
      settings: OpenFcn=open_system([gcb '/Actuator'],'mask')
      mask Help: eval('openHelp(222)')
      mask Display: image(imread('State.png'))
  STATE_Mazda_RX8_2_bus : Subsystem  Tag=actuator/StatePort  Priority=0  LoadFcn=load('PreScanStateActuatorData.mat')  mask(PreScan Sink Block: State){}
      mask help:
      | The Actor State contains a vector signal of size (9x1), containing the following signals:
      |
      | -  Position    	(x,y,z)             	[m]
      | -  Velocity    	(vx,vy,vz)         	[m/s]
      | -  Angles       	(Roll, Pitch, Yaw)	[rad]
      |
      | The Actor state is defined in the global axis system.
      | The state is superponed on the Initial position defined in the GUI.
      |
      | For more information, please click Help.
      settings: OpenFcn=open_system([gcb '/Actuator'],'mask')
      mask Help: eval('openHelp(222)')
      mask Display: image(imread('State.png'))
  STATE_Mazda_RX8_3_bus : Subsystem  Tag=actuator/StatePort  Priority=0  LoadFcn=load('PreScanStateActuatorData.mat')  mask(PreScan Sink Block: State){}
      mask help:
      | The Actor State contains a vector signal of size (9x1), containing the following signals:
      |
      | -  Position    	(x,y,z)             	[m]
      | -  Velocity    	(vx,vy,vz)         	[m/s]
      | -  Angles       	(Roll, Pitch, Yaw)	[rad]
      |
      | The Actor state is defined in the global axis system.
      | The state is superponed on the Initial position defined in the GUI.
      |
      | For more information, please click Help.
      settings: OpenFcn=open_system([gcb '/Actuator'],'mask')
      mask Help: eval('openHelp(222)')
      mask Display: image(imread('State.png'))
  STATE_Nissan_Cabstar_1_bus : Subsystem  Tag=actuator/StatePort  Priority=0  LoadFcn=load('PreScanStateActuatorData.mat')  mask(PreScan Sink Block: State){}
      mask help:
      | The Actor State contains a vector signal of size (9x1), containing the following signals:
      |
      | -  Position    	(x,y,z)             	[m]
      | -  Velocity    	(vx,vy,vz)         	[m/s]
      | -  Angles       	(Roll, Pitch, Yaw)	[rad]
      |
      | The Actor state is defined in the global axis system.
      | The state is superponed on the Initial position defined in the GUI.
      |
      | For more information, please click Help.
      settings: OpenFcn=open_system([gcb '/Actuator'],'mask')
      mask Help: eval('openHelp(222)')
      mask Display: image(imread('State.png'))
  STATE_Sphere_1_bus : Subsystem  Tag=actuator/StatePort  Priority=0  LoadFcn=load('PreScanStateActuatorData.mat')  mask(PreScan Sink Block: State){}
      mask help:
      | The Actor State contains a vector signal of size (9x1), containing the following signals:
      |
      | -  Position    	(x,y,z)             	[m]
      | -  Velocity    	(vx,vy,vz)         	[m/s]
      | -  Angles       	(Roll, Pitch, Yaw)	[rad]
      |
      | The Actor state is defined in the global axis system.
      | The state is superponed on the Initial position defined in the GUI.
      |
      | For more information, please click Help.
      settings: OpenFcn=open_system([gcb '/Actuator'],'mask')
      mask Help: eval('openHelp(222)')
      mask Display: image(imread('State.png'))
  STATE_Toyota_Previa_1_bus : Subsystem  Tag=actuator/StatePort  Priority=0  LoadFcn=load('PreScanStateActuatorData.mat')  mask(PreScan Sink Block: State){}
      mask help:
      | The Actor State contains a vector signal of size (9x1), containing the following signals:
      |
      | -  Position    	(x,y,z)             	[m]
      | -  Velocity    	(vx,vy,vz)         	[m/s]
      | -  Angles       	(Roll, Pitch, Yaw)	[rad]
      |
      | The Actor state is defined in the global axis system.
      | The state is superponed on the Initial position defined in the GUI.
      |
      | For more information, please click Help.
      settings: OpenFcn=open_system([gcb '/Actuator'],'mask')
      mask Help: eval('openHelp(222)')
      mask Display: image(imread('State.png'))
  STATE_Toyota_Previa_2_bus : Subsystem  Tag=actuator/StatePort  Priority=0  LoadFcn=load('PreScanStateActuatorData.mat')  mask(PreScan Sink Block: State){}
      mask help:
      | The Actor State contains a vector signal of size (9x1), containing the following signals:
      |
      | -  Position    	(x,y,z)             	[m]
      | -  Velocity    	(vx,vy,vz)         	[m/s]
      | -  Angles       	(Roll, Pitch, Yaw)	[rad]
      |
      | The Actor state is defined in the global axis system.
      | The state is superponed on the Initial position defined in the GUI.
      |
      | For more information, please click Help.
      settings: OpenFcn=open_system([gcb '/Actuator'],'mask')
      mask Help: eval('openHelp(222)')
      mask Display: image(imread('State.png'))
  STATE_Toyota_Yaris_1_bus : Subsystem  Tag=actuator/StatePort  Priority=0  LoadFcn=load('PreScanStateActuatorData.mat')  mask(PreScan Sink Block: State){}
      mask help:
      | The Actor State contains a vector signal of size (9x1), containing the following signals:
      |
      | -  Position    	(x,y,z)             	[m]
      | -  Velocity    	(vx,vy,vz)         	[m/s]
      | -  Angles       	(Roll, Pitch, Yaw)	[rad]
      |
      | The Actor state is defined in the global axis system.
      | The state is superponed on the Initial position defined in the GUI.
      |
      | For more information, please click Help.
      settings: OpenFcn=open_system([gcb '/Actuator'],'mask')
      mask Help: eval('openHelp(222)')
      mask Display: image(imread('State.png'))
  ScenarioEngine : Subsystem  Tag=PreScanOpenScenarioBlock  Priority=10  LoadFcn=load PrescanSynchronizeData  mask(PreScan Simulation Core Block){TimeStep=1/100}
      mask prompts: TimeStep "Timestep [s]"
      mask help:
      | Please do not remove this block from the PreScan compilation sheet,
      | as it contains essential configuration parameters for a PreScan simulation.
      settings: DeleteFcn=PreScanBlockDeleteFcn;
      mask Display: image(imread('prescanlogo.ico'))
  Sphere_1 : Subsystem  Tag=WorldObjectSubSystem  InitFcn=UniqueId = '277';
      mask init:
      | imagePath=which('Sphere.jpg');
      mask Display: image(imread(imagePath));color('white');text(0, 0, ' ID=2\n')
  SteeringColumn_pivot_Audi_A8_1 : Subsystem  Tag=Actuator  Priority=0  LoadFcn=load('PrescanPoseData');load('PrescanXYZData');load('PreScanRPYData')
      mask help:
      | The VisuJoint block provides a way to adapt the location and orientation of a part of an object.
      |
      | For more information, please click Help.
      settings: OpenFcn=open_system([gcb '/Actuator'],'mask')
      mask Display: image(imread('Joint.png'))
  SteeringWheel_pivot_Audi_A8_1 : Subsystem  Tag=Actuator  Priority=0  LoadFcn=load('PrescanPoseData');load('PrescanXYZData');load('PreScanRPYData')
      mask help:
      | The VisuJoint block provides a way to adapt the location and orientation of a part of an object.
      |
      | For more information, please click Help.
      settings: OpenFcn=open_system([gcb '/Actuator'],'mask')
      mask Display: image(imread('Joint.png'))
  Synchronizer : Subsystem  Tag=PreScanSynchronizer  Priority=20  LoadFcn=load PrescanSynchronizeData  mask(PreScan Simulation Core Block){TimeStep=1/100}
      mask prompts: TimeStep "Timestep [s]"
      mask help:
      | Please do not remove this block from the PreScan compilation sheet,
      | as it contains essential configuration parameters for a PreScan simulation.
      settings: DeleteFcn=PreScanBlockDeleteFcn;
      mask Display: image(imread('prescanlogo.ico'))
  Toyota_Previa_1 : Subsystem  Tag=WorldObjectSubSystem  InitFcn=UniqueId = '1688';
      mask init:
      | modelPath = GenericModelHelper.getGenericModelFilePath('ModelDepo','Vehicles\Toyota_Previa\Toyota_Previa.pgmb','93e58f95175b34f6ce91a88cdfe55b40');imagePath = GenericModelHelper.getCompilationPicture(modelPath, 'Toyota_Previa_HighPoly.png');
      mask Display: image(imread(imagePath));color('white');text(0, 0, ' ID=838\n')
  Toyota_Previa_2 : Subsystem  Tag=WorldObjectSubSystem  InitFcn=UniqueId = '1970';
      mask init: same as TSR_Scenario_001_cs/Toyota_Previa_1
      mask Display: image(imread(imagePath));color('white');text(0, 0, ' ID=1008\n')
  Toyota_Yaris_1 : Subsystem  Tag=WorldObjectSubSystem  InitFcn=UniqueId = '1961';
      mask init:
      | modelPath = GenericModelHelper.getGenericModelFilePath('ModelDepo','Vehicles\Toyota_Yaris\Toyota_Yaris.pgmb','3ea2b9be97d70b5ca322b210574befd9');imagePath = GenericModelHelper.getCompilationPicture(modelPath, 'Toyota_Yaris_HighPoly.png');
      mask Display: image(imread(imagePath));color('white');text(0, 0, ' ID=1005\n')
  VISUColorRegion_Exterior_Audi_A8_2 : Subsystem  Tag=actuator/ColorRegion  Priority=0  LoadFcn=load('PrescanColorData')  mask(PreScan Sink Block: VisuTextureColor){}
      mask help:
      | The VisuTextureColor block provides a way to adapt the color of a vehicle.
      |
      | For more information, please click Help.
      settings: OpenFcn=open_system([gcb '/Actuator'],'mask')
      mask Help: eval('openHelp(230)')
      mask Display: image(imread('TextureColor.png'))
  VISUColorRegion_Exterior_BMW_Z3_1 : Subsystem  Tag=actuator/ColorRegion  Priority=0  LoadFcn=load('PrescanColorData')  mask(PreScan Sink Block: VisuTextureColor){}
      mask help:
      | The VisuTextureColor block provides a way to adapt the color of a vehicle.
      |
      | For more information, please click Help.
      settings: OpenFcn=open_system([gcb '/Actuator'],'mask')
      mask Help: eval('openHelp(230)')
      mask Display: image(imread('TextureColor.png'))
  VISUColorRegion_Exterior_BMW_Z3_2 : Subsystem  Tag=actuator/ColorRegion  Priority=0  LoadFcn=load('PrescanColorData')  mask(PreScan Sink Block: VisuTextureColor){}
      mask help:
      | The VisuTextureColor block provides a way to adapt the color of a vehicle.
      |
      | For more information, please click Help.
      settings: OpenFcn=open_system([gcb '/Actuator'],'mask')
      mask Help: eval('openHelp(230)')
      mask Display: image(imread('TextureColor.png'))
  VISUColorRegion_Exterior_Citroen_C3_1 : Subsystem  Tag=actuator/ColorRegion  Priority=0  LoadFcn=load('PrescanColorData')  mask(PreScan Sink Block: VisuTextureColor){}
      mask help:
      | The VisuTextureColor block provides a way to adapt the color of a vehicle.
      |
      | For more information, please click Help.
      settings: OpenFcn=open_system([gcb '/Actuator'],'mask')
      mask Help: eval('openHelp(230)')
      mask Display: image(imread('TextureColor.png'))
  VISUColorRegion_Exterior_Citroen_C3_2 : Subsystem  Tag=actuator/ColorRegion  Priority=0  LoadFcn=load('PrescanColorData')  mask(PreScan Sink Block: VisuTextureColor){}
      mask help:
      | The VisuTextureColor block provides a way to adapt the color of a vehicle.
      |
      | For more information, please click Help.
      settings: OpenFcn=open_system([gcb '/Actuator'],'mask')
      mask Help: eval('openHelp(230)')
      mask Display: image(imread('TextureColor.png'))
  VISUColorRegion_Exterior_Citroen_C3_3 : Subsystem  Tag=actuator/ColorRegion  Priority=0  LoadFcn=load('PrescanColorData')  mask(PreScan Sink Block: VisuTextureColor){}
      mask help:
      | The VisuTextureColor block provides a way to adapt the color of a vehicle.
      |
      | For more information, please click Help.
      settings: OpenFcn=open_system([gcb '/Actuator'],'mask')
      mask Help: eval('openHelp(230)')
      mask Display: image(imread('TextureColor.png'))
  VISUColorRegion_Exterior_Citroen_C3_4 : Subsystem  Tag=actuator/ColorRegion  Priority=0  LoadFcn=load('PrescanColorData')  mask(PreScan Sink Block: VisuTextureColor){}
      mask help:
      | The VisuTextureColor block provides a way to adapt the color of a vehicle.
      |
      | For more information, please click Help.
      settings: OpenFcn=open_system([gcb '/Actuator'],'mask')
      mask Help: eval('openHelp(230)')
      mask Display: image(imread('TextureColor.png'))
  VISUColorRegion_Exterior_Fiat_Bravo_1 : Subsystem  Tag=actuator/ColorRegion  Priority=0  LoadFcn=load('PrescanColorData')  mask(PreScan Sink Block: VisuTextureColor){}
      mask help:
      | The VisuTextureColor block provides a way to adapt the color of a vehicle.
      |
      | For more information, please click Help.
      settings: OpenFcn=open_system([gcb '/Actuator'],'mask')
      mask Help: eval('openHelp(230)')
      mask Display: image(imread('TextureColor.png'))
  VISUColorRegion_Exterior_Ford_Fiesta_1 : Subsystem  Tag=actuator/ColorRegion  Priority=0  LoadFcn=load('PrescanColorData')  mask(PreScan Sink Block: VisuTextureColor){}
      mask help:
      | The VisuTextureColor block provides a way to adapt the color of a vehicle.
      |
      | For more information, please click Help.
      settings: OpenFcn=open_system([gcb '/Actuator'],'mask')
      mask Help: eval('openHelp(230)')
      mask Display: image(imread('TextureColor.png'))
  VISUColorRegion_Exterior_Mazda_RX8_1 : Subsystem  Tag=actuator/ColorRegion  Priority=0  LoadFcn=load('PrescanColorData')  mask(PreScan Sink Block: VisuTextureColor){}
      mask help:
      | The VisuTextureColor block provides a way to adapt the color of a vehicle.
      |
      | For more information, please click Help.
      settings: OpenFcn=open_system([gcb '/Actuator'],'mask')
      mask Help: eval('openHelp(230)')
      mask Display: image(imread('TextureColor.png'))
  VISUColorRegion_Exterior_Mazda_RX8_2 : Subsystem  Tag=actuator/ColorRegion  Priority=0  LoadFcn=load('PrescanColorData')  mask(PreScan Sink Block: VisuTextureColor){}
      mask help:
      | The VisuTextureColor block provides a way to adapt the color of a vehicle.
      |
      | For more information, please click Help.
      settings: OpenFcn=open_system([gcb '/Actuator'],'mask')
      mask Help: eval('openHelp(230)')
      mask Display: image(imread('TextureColor.png'))
  VISUColorRegion_Exterior_Mazda_RX8_3 : Subsystem  Tag=actuator/ColorRegion  Priority=0  LoadFcn=load('PrescanColorData')  mask(PreScan Sink Block: VisuTextureColor){}
      mask help:
      | The VisuTextureColor block provides a way to adapt the color of a vehicle.
      |
      | For more information, please click Help.
      settings: OpenFcn=open_system([gcb '/Actuator'],'mask')
      mask Help: eval('openHelp(230)')
      mask Display: image(imread('TextureColor.png'))
  VISUColorRegion_Exterior_Nissan_Cabstar_1 : Subsystem  Tag=actuator/ColorRegion  Priority=0  LoadFcn=load('PrescanColorData')  mask(PreScan Sink Block: VisuTextureColor){}
      mask help:
      | The VisuTextureColor block provides a way to adapt the color of a vehicle.
      |
      | For more information, please click Help.
      settings: OpenFcn=open_system([gcb '/Actuator'],'mask')
      mask Help: eval('openHelp(230)')
      mask Display: image(imread('TextureColor.png'))
  VISUColorRegion_Exterior_Toyota_Previa_1 : Subsystem  Tag=actuator/ColorRegion  Priority=0  LoadFcn=load('PrescanColorData')  mask(PreScan Sink Block: VisuTextureColor){}
      mask help:
      | The VisuTextureColor block provides a way to adapt the color of a vehicle.
      |
      | For more information, please click Help.
      settings: OpenFcn=open_system([gcb '/Actuator'],'mask')
      mask Help: eval('openHelp(230)')
      mask Display: image(imread('TextureColor.png'))
  VISUColorRegion_Exterior_Toyota_Previa_2 : Subsystem  Tag=actuator/ColorRegion  Priority=0  LoadFcn=load('PrescanColorData')  mask(PreScan Sink Block: VisuTextureColor){}
      mask help:
      | The VisuTextureColor block provides a way to adapt the color of a vehicle.
      |
      | For more information, please click Help.
      settings: OpenFcn=open_system([gcb '/Actuator'],'mask')
      mask Help: eval('openHelp(230)')
      mask Display: image(imread('TextureColor.png'))
  VISUColorRegion_Exterior_Toyota_Yaris_1 : Subsystem  Tag=actuator/ColorRegion  Priority=0  LoadFcn=load('PrescanColorData')  mask(PreScan Sink Block: VisuTextureColor){}
      mask help:
      | The VisuTextureColor block provides a way to adapt the color of a vehicle.
      |
      | For more information, please click Help.
      settings: OpenFcn=open_system([gcb '/Actuator'],'mask')
      mask Help: eval('openHelp(230)')
      mask Display: image(imread('TextureColor.png'))
  VISUMatrixSignLights_HighwayOverhang_1 : Subsystem  Tag=actuator/VisuMatrixSignLights  Priority=0  mask(PreScan Sink Block: VisuMatrixSignLights){UniqueID=1876, ColorsObjectQuery=, Colors=[]}
      mask prompts: UniqueID "Parent Unique Identifier"; ColorsObjectQuery "Query for Color Object"; Colors "Matrix of colors"
      mask help:
      | The VisuMatrixSignLights block provides a way to switch the lights on the matrix sign board on or off
      |
      | For more information, please click Help.
      settings: OpenFcn=open_system([gcb '/Actuator'],'mask')
      mask Help: eval('openHelp(732)')
      mask Display: image(imread('RearLight.png'))
  VISUMatrixSignLights_HighwayOverhang_2 : Subsystem  Tag=actuator/VisuMatrixSignLights  Priority=0  mask(PreScan Sink Block: VisuMatrixSignLights){UniqueID=1877, ColorsObjectQuery=, Colors=[]}
      mask prompts: UniqueID "Parent Unique Identifier"; ColorsObjectQuery "Query for Color Object"; Colors "Matrix of colors"
      mask help:
      | The VisuMatrixSignLights block provides a way to switch the lights on the matrix sign board on or off
      |
      | For more information, please click Help.
      settings: OpenFcn=open_system([gcb '/Actuator'],'mask')
      mask Help: eval('openHelp(732)')
      mask Display: image(imread('RearLight.png'))
  VISUMatrixSignLights_HighwayOverhang_3 : Subsystem  Tag=actuator/VisuMatrixSignLights  Priority=0  mask(PreScan Sink Block: VisuMatrixSignLights){UniqueID=1890, ColorsObjectQuery=, Colors=[]}
      mask prompts: UniqueID "Parent Unique Identifier"; ColorsObjectQuery "Query for Color Object"; Colors "Matrix of colors"
      mask help:
      | The VisuMatrixSignLights block provides a way to switch the lights on the matrix sign board on or off
      |
      | For more information, please click Help.
      settings: OpenFcn=open_system([gcb '/Actuator'],'mask')
      mask Help: eval('openHelp(732)')
      mask Display: image(imread('RearLight.png'))
  VISUMatrixSignLights_HighwayOverhang_4 : Subsystem  Tag=actuator/VisuMatrixSignLights  Priority=0  mask(PreScan Sink Block: VisuMatrixSignLights){UniqueID=1898, ColorsObjectQuery=, Colors=[]}
      mask prompts: UniqueID "Parent Unique Identifier"; ColorsObjectQuery "Query for Color Object"; Colors "Matrix of colors"
      mask help:
      | The VisuMatrixSignLights block provides a way to switch the lights on the matrix sign board on or off
      |
      | For more information, please click Help.
      settings: OpenFcn=open_system([gcb '/Actuator'],'mask')
      mask Help: eval('openHelp(732)')
      mask Display: image(imread('RearLight.png'))
  VISUMatrixSignLights_HighwayOverhang_5 : Subsystem  Tag=actuator/VisuMatrixSignLights  Priority=0  mask(PreScan Sink Block: VisuMatrixSignLights){UniqueID=1909, ColorsObjectQuery=, Colors=[]}
      mask prompts: UniqueID "Parent Unique Identifier"; ColorsObjectQuery "Query for Color Object"; Colors "Matrix of colors"
      mask help:
      | The VisuMatrixSignLights block provides a way to switch the lights on the matrix sign board on or off
      |
      | For more information, please click Help.
      settings: OpenFcn=open_system([gcb '/Actuator'],'mask')
      mask Help: eval('openHelp(732)')
      mask Display: image(imread('RearLight.png'))
  VISUMatrixSignLights_HighwayOverhang_6 : Subsystem  Tag=actuator/VisuMatrixSignLights  Priority=0  mask(PreScan Sink Block: VisuMatrixSignLights){UniqueID=1914, ColorsObjectQuery=, Colors=[]}
      mask prompts: UniqueID "Parent Unique Identifier"; ColorsObjectQuery "Query for Color Object"; Colors "Matrix of colors"
      mask help:
      | The VisuMatrixSignLights block provides a way to switch the lights on the matrix sign board on or off
      |
      | For more information, please click Help.
      settings: OpenFcn=open_system([gcb '/Actuator'],'mask')
      mask Help: eval('openHelp(732)')
      mask Display: image(imread('RearLight.png'))
  VISUMatrixSign_HighwayOverhang_1 : Subsystem  Tag=actuator/VisuMatrixSign  Priority=0  mask(PreScan Sink Block: VisuMatrixSign){UniqueID=1876, ResourceList={'3' 'InformationSign\MatrixSign_Empty.png' '4' 'InformationSign\MatrixSign_End.png' '5' 'InformationSign\MatrixSign_GreenArrow.png' '6' 'InformationSign\MatrixSign_RedCross.png' '7' 'InformationSign\MatrixSign_Speed_50.png' '8' 'InformationSign\MatrixSign_Speed_70.png' '9' 'InformationSign\MatrixSign_Speed_90.png' '10' 'InformationSign\MatrixSign_Speed_120.png' '11' 'InformationSign\MatrixSign_Speed_130.png' '12' 'InformationSign\information.png' '13' 'InformationSign\Empty.jpg' }, PivotName=}
      mask prompts: UniqueID "Parent Unique Identifier (auto-generated)"; ResourceList "Resource List (auto-generated)"; PivotName "Name of pivot (auto-generated)"
      mask help:
      | The VisuMatrixSign block provides a way to adapt the texture of the plates connected to an overhang, based on Resource IDs of the texture files.
      |
      | For more information, please click Help.
      settings: OpenFcn=open_system([gcb '/Actuator'],'mask')
      mask Help: eval('openHelp(733)')
      mask Display: image(imread('HighwaySpeedMatrix.png'))
  VISUMatrixSign_HighwayOverhang_2 : Subsystem  Tag=actuator/VisuMatrixSign  Priority=0  mask(PreScan Sink Block: VisuMatrixSign){UniqueID=1877, ResourceList={'3' 'InformationSign\MatrixSign_Empty.png' '4' 'InformationSign\MatrixSign_End.png' '5' 'InformationSign\MatrixSign_GreenArrow.png' '6' 'InformationSign\MatrixSign_RedCross.png' '7' 'InformationSign\MatrixSign_Speed_50.png' '8' 'InformationSign\MatrixSign_Speed_70.png' '9' 'InformationSign\MatrixSign_Speed_90.png' '10' 'InformationSign\MatrixSign_Speed_120.png' '11' 'InformationSign\MatrixSign_Speed_130.png' '12' 'InformationSign\information.png' '13' 'InformationSign\Empty.jpg' }, PivotName=}
      mask prompts: UniqueID "Parent Unique Identifier (auto-generated)"; ResourceList "Resource List (auto-generated)"; PivotName "Name of pivot (auto-generated)"
      mask help:
      | The VisuMatrixSign block provides a way to adapt the texture of the plates connected to an overhang, based on Resource IDs of the texture files.
      |
      | For more information, please click Help.
      settings: OpenFcn=open_system([gcb '/Actuator'],'mask')
      mask Help: eval('openHelp(733)')
      mask Display: image(imread('HighwaySpeedMatrix.png'))
  VISUMatrixSign_HighwayOverhang_3 : Subsystem  Tag=actuator/VisuMatrixSign  Priority=0  mask(PreScan Sink Block: VisuMatrixSign){UniqueID=1890, ResourceList={'3' 'InformationSign\MatrixSign_Empty.png' '4' 'InformationSign\MatrixSign_End.png' '5' 'InformationSign\MatrixSign_GreenArrow.png' '6' 'InformationSign\MatrixSign_RedCross.png' '7' 'InformationSign\MatrixSign_Speed_50.png' '8' 'InformationSign\MatrixSign_Speed_70.png' '9' 'InformationSign\MatrixSign_Speed_90.png' '10' 'InformationSign\MatrixSign_Speed_120.png' '11' 'InformationSign\MatrixSign_Speed_130.png' '12' 'InformationSign\information.png' '13' 'InformationSign\Empty.jpg' }, PivotName=}
      mask prompts: UniqueID "Parent Unique Identifier (auto-generated)"; ResourceList "Resource List (auto-generated)"; PivotName "Name of pivot (auto-generated)"
      mask help:
      | The VisuMatrixSign block provides a way to adapt the texture of the plates connected to an overhang, based on Resource IDs of the texture files.
      |
      | For more information, please click Help.
      settings: OpenFcn=open_system([gcb '/Actuator'],'mask')
      mask Help: eval('openHelp(733)')
      mask Display: image(imread('HighwaySpeedMatrix.png'))
  VISUMatrixSign_HighwayOverhang_4 : Subsystem  Tag=actuator/VisuMatrixSign  Priority=0  mask(PreScan Sink Block: VisuMatrixSign){UniqueID=1898, ResourceList={'3' 'InformationSign\MatrixSign_Empty.png' '4' 'InformationSign\MatrixSign_End.png' '5' 'InformationSign\MatrixSign_GreenArrow.png' '6' 'InformationSign\MatrixSign_RedCross.png' '7' 'InformationSign\MatrixSign_Speed_50.png' '8' 'InformationSign\MatrixSign_Speed_70.png' '9' 'InformationSign\MatrixSign_Speed_90.png' '10' 'InformationSign\MatrixSign_Speed_120.png' '11' 'InformationSign\MatrixSign_Speed_130.png' '12' 'InformationSign\information.png' '13' 'InformationSign\Empty.jpg' }, PivotName=}
      mask prompts: UniqueID "Parent Unique Identifier (auto-generated)"; ResourceList "Resource List (auto-generated)"; PivotName "Name of pivot (auto-generated)"
      mask help:
      | The VisuMatrixSign block provides a way to adapt the texture of the plates connected to an overhang, based on Resource IDs of the texture files.
      |
      | For more information, please click Help.
      settings: OpenFcn=open_system([gcb '/Actuator'],'mask')
      mask Help: eval('openHelp(733)')
      mask Display: image(imread('HighwaySpeedMatrix.png'))
  VISUMatrixSign_HighwayOverhang_5 : Subsystem  Tag=actuator/VisuMatrixSign  Priority=0  mask(PreScan Sink Block: VisuMatrixSign){UniqueID=1909, ResourceList={'3' 'InformationSign\MatrixSign_Empty.png' '4' 'InformationSign\MatrixSign_End.png' '5' 'InformationSign\MatrixSign_GreenArrow.png' '6' 'InformationSign\MatrixSign_RedCross.png' '7' 'InformationSign\MatrixSign_Speed_50.png' '8' 'InformationSign\MatrixSign_Speed_70.png' '9' 'InformationSign\MatrixSign_Speed_90.png' '10' 'InformationSign\MatrixSign_Speed_120.png' '11' 'InformationSign\MatrixSign_Speed_130.png' '12' 'InformationSign\information.png' '13' 'InformationSign\Empty.jpg' }, PivotName=}
      mask prompts: UniqueID "Parent Unique Identifier (auto-generated)"; ResourceList "Resource List (auto-generated)"; PivotName "Name of pivot (auto-generated)"
      mask help:
      | The VisuMatrixSign block provides a way to adapt the texture of the plates connected to an overhang, based on Resource IDs of the texture files.
      |
      | For more information, please click Help.
      settings: OpenFcn=open_system([gcb '/Actuator'],'mask')
      mask Help: eval('openHelp(733)')
      mask Display: image(imread('HighwaySpeedMatrix.png'))
  VISUMatrixSign_HighwayOverhang_6 : Subsystem  Tag=actuator/VisuMatrixSign  Priority=0  mask(PreScan Sink Block: VisuMatrixSign){UniqueID=1914, ResourceList={'3' 'InformationSign\MatrixSign_Empty.png' '4' 'InformationSign\MatrixSign_End.png' '5' 'InformationSign\MatrixSign_GreenArrow.png' '6' 'InformationSign\MatrixSign_RedCross.png' '7' 'InformationSign\MatrixSign_Speed_50.png' '8' 'InformationSign\MatrixSign_Speed_70.png' '9' 'InformationSign\MatrixSign_Speed_90.png' '10' 'InformationSign\MatrixSign_Speed_120.png' '11' 'InformationSign\MatrixSign_Speed_130.png' '12' 'InformationSign\information.png' '13' 'InformationSign\Empty.jpg' }, PivotName=}
      mask prompts: UniqueID "Parent Unique Identifier (auto-generated)"; ResourceList "Resource List (auto-generated)"; PivotName "Name of pivot (auto-generated)"
      mask help:
      | The VisuMatrixSign block provides a way to adapt the texture of the plates connected to an overhang, based on Resource IDs of the texture files.
      |
      | For more information, please click Help.
      settings: OpenFcn=open_system([gcb '/Actuator'],'mask')
      mask Help: eval('openHelp(733)')
      mask Display: image(imread('HighwaySpeedMatrix.png'))
  VISUMatrixSign_HighwayOverhang_7 : Subsystem  Tag=actuator/VisuMatrixSign  Priority=0  mask(PreScan Sink Block: VisuMatrixSign){UniqueID=2612, ResourceList={'3' 'InformationSign\MatrixSign_Empty.png' '4' 'InformationSign\MatrixSign_End.png' '5' 'InformationSign\MatrixSign_GreenArrow.png' '6' 'InformationSign\MatrixSign_RedCross.png' '7' 'InformationSign\MatrixSign_Speed_50.png' '8' 'InformationSign\MatrixSign_Speed_70.png' '9' 'InformationSign\MatrixSign_Speed_90.png' '10' 'InformationSign\MatrixSign_Speed_120.png' '11' 'InformationSign\MatrixSign_Speed_130.png' '12' 'InformationSign\information.png' '13' 'InformationSign\Empty.jpg' }, PivotName=}
      mask prompts: UniqueID "Parent Unique Identifier (auto-generated)"; ResourceList "Resource List (auto-generated)"; PivotName "Name of pivot (auto-generated)"
      mask help:
      | The VisuMatrixSign block provides a way to adapt the texture of the plates connected to an overhang, based on Resource IDs of the texture files.
      |
      | For more information, please click Help.
      settings: OpenFcn=open_system([gcb '/Actuator'],'mask')
      mask Help: eval('openHelp(733)')
      mask Display: image(imread('HighwaySpeedMatrix.png'))
  WheelL0_Actros_2541_2 : Subsystem  Tag=Actuator  Priority=0  LoadFcn=load('PrescanPoseData');load('PrescanXYZData');load('PreScanRPYData')
      mask help:
      | The VisuJoint block provides a way to adapt the location and orientation of a part of an object.
      |
      | For more information, please click Help.
      settings: OpenFcn=open_system([gcb '/Actuator'],'mask')
      mask Display: image(imread('Joint.png'))
  WheelL0_Audi_A8_1 : Subsystem  Tag=Actuator  Priority=0  LoadFcn=load('PrescanPoseData');load('PrescanXYZData');load('PreScanRPYData')
      mask help:
      | The VisuJoint block provides a way to adapt the location and orientation of a part of an object.
      |
      | For more information, please click Help.
      settings: OpenFcn=open_system([gcb '/Actuator'],'mask')
      mask Display: image(imread('Joint.png'))
  WheelL0_Audi_A8_2 : Subsystem  Tag=Actuator  Priority=0  LoadFcn=load('PrescanPoseData');load('PrescanXYZData');load('PreScanRPYData')
      mask help:
      | The VisuJoint block provides a way to adapt the location and orientation of a part of an object.
      |
      | For more information, please click Help.
      settings: OpenFcn=open_system([gcb '/Actuator'],'mask')
      mask Display: image(imread('Joint.png'))
  WheelL0_BMW_Z3_1 : Subsystem  Tag=Actuator  Priority=0  LoadFcn=load('PrescanPoseData');load('PrescanXYZData');load('PreScanRPYData')
      mask help:
      | The VisuJoint block provides a way to adapt the location and orientation of a part of an object.
      |
      | For more information, please click Help.
      settings: OpenFcn=open_system([gcb '/Actuator'],'mask')
      mask Display: image(imread('Joint.png'))
  WheelL0_BMW_Z3_2 : Subsystem  Tag=Actuator  Priority=0  LoadFcn=load('PrescanPoseData');load('PrescanXYZData');load('PreScanRPYData')
      mask help:
      | The VisuJoint block provides a way to adapt the location and orientation of a part of an object.
      |
      | For more information, please click Help.
      settings: OpenFcn=open_system([gcb '/Actuator'],'mask')
      mask Display: image(imread('Joint.png'))
  WheelL0_Citroen_C3_1 : Subsystem  Tag=Actuator  Priority=0  LoadFcn=load('PrescanPoseData');load('PrescanXYZData');load('PreScanRPYData')
      mask help:
      | The VisuJoint block provides a way to adapt the location and orientation of a part of an object.
      |
      | For more information, please click Help.
      settings: OpenFcn=open_system([gcb '/Actuator'],'mask')
      mask Display: image(imread('Joint.png'))
  WheelL0_Citroen_C3_2 : Subsystem  Tag=Actuator  Priority=0  LoadFcn=load('PrescanPoseData');load('PrescanXYZData');load('PreScanRPYData')
      mask help:
      | The VisuJoint block provides a way to adapt the location and orientation of a part of an object.
      |
      | For more information, please click Help.
      settings: OpenFcn=open_system([gcb '/Actuator'],'mask')
      mask Display: image(imread('Joint.png'))
  WheelL0_Citroen_C3_3 : Subsystem  Tag=Actuator  Priority=0  LoadFcn=load('PrescanPoseData');load('PrescanXYZData');load('PreScanRPYData')
      mask help:
      | The VisuJoint block provides a way to adapt the location and orientation of a part of an object.
      |
      | For more information, please click Help.
      settings: OpenFcn=open_system([gcb '/Actuator'],'mask')
      mask Display: image(imread('Joint.png'))
  WheelL0_Citroen_C3_4 : Subsystem  Tag=Actuator  Priority=0  LoadFcn=load('PrescanPoseData');load('PrescanXYZData');load('PreScanRPYData')
      mask help:
      | The VisuJoint block provides a way to adapt the location and orientation of a part of an object.
      |
      | For more information, please click Help.
      settings: OpenFcn=open_system([gcb '/Actuator'],'mask')
      mask Display: image(imread('Joint.png'))
  WheelL0_Fiat_Bravo_1 : Subsystem  Tag=Actuator  Priority=0  LoadFcn=load('PrescanPoseData');load('PrescanXYZData');load('PreScanRPYData')
      mask help:
      | The VisuJoint block provides a way to adapt the location and orientation of a part of an object.
      |
      | For more information, please click Help.
      settings: OpenFcn=open_system([gcb '/Actuator'],'mask')
      mask Display: image(imread('Joint.png'))
  WheelL0_Fiat_Bravo_2 : Subsystem  Tag=Actuator  Priority=0  LoadFcn=load('PrescanPoseData');load('PrescanXYZData');load('PreScanRPYData')
      mask help:
      | The VisuJoint block provides a way to adapt the location and orientation of a part of an object.
      |
      | For more information, please click Help.
      settings: OpenFcn=open_system([gcb '/Actuator'],'mask')
      mask Display: image(imread('Joint.png'))
  WheelL0_Ford_Fiesta_1 : Subsystem  Tag=Actuator  Priority=0  LoadFcn=load('PrescanPoseData');load('PrescanXYZData');load('PreScanRPYData')
      mask help:
      | The VisuJoint block provides a way to adapt the location and orientation of a part of an object.
      |
      | For more information, please click Help.
      settings: OpenFcn=open_system([gcb '/Actuator'],'mask')
      mask Display: image(imread('Joint.png'))
  WheelL0_Mazda_RX8_2 : Subsystem  Tag=Actuator  Priority=0  LoadFcn=load('PrescanPoseData');load('PrescanXYZData');load('PreScanRPYData')
      mask help:
      | The VisuJoint block provides a way to adapt the location and orientation of a part of an object.
      |
      | For more information, please click Help.
      settings: OpenFcn=open_system([gcb '/Actuator'],'mask')
      mask Display: image(imread('Joint.png'))
  WheelL0_Mazda_RX8_3 : Subsystem  Tag=Actuator  Priority=0  LoadFcn=load('PrescanPoseData');load('PrescanXYZData');load('PreScanRPYData')
      mask help:
      | The VisuJoint block provides a way to adapt the location and orientation of a part of an object.
      |
      | For more information, please click Help.
      settings: OpenFcn=open_system([gcb '/Actuator'],'mask')
      mask Display: image(imread('Joint.png'))
  WheelL0_Toyota_Previa_2 : Subsystem  Tag=Actuator  Priority=0  LoadFcn=load('PrescanPoseData');load('PrescanXYZData');load('PreScanRPYData')
      mask help:
      | The VisuJoint block provides a way to adapt the location and orientation of a part of an object.
      |
      | For more information, please click Help.
      settings: OpenFcn=open_system([gcb '/Actuator'],'mask')
      mask Display: image(imread('Joint.png'))
  WheelL0_Toyota_Yaris_1 : Subsystem  Tag=Actuator  Priority=0  LoadFcn=load('PrescanPoseData');load('PrescanXYZData');load('PreScanRPYData')
      mask help:
      | The VisuJoint block provides a way to adapt the location and orientation of a part of an object.
      |
      | For more information, please click Help.
      settings: OpenFcn=open_system([gcb '/Actuator'],'mask')
      mask Display: image(imread('Joint.png'))
  WheelL1_Actros_2541_2 : Subsystem  Tag=Actuator  Priority=0  LoadFcn=load('PrescanPoseData');load('PrescanXYZData');load('PreScanRPYData')
      mask help:
      | The VisuJoint block provides a way to adapt the location and orientation of a part of an object.
      |
      | For more information, please click Help.
      settings: OpenFcn=open_system([gcb '/Actuator'],'mask')
      mask Display: image(imread('Joint.png'))
  WheelL1_Audi_A8_1 : Subsystem  Tag=Actuator  Priority=0  LoadFcn=load('PrescanPoseData');load('PrescanXYZData');load('PreScanRPYData')
      mask help:
      | The VisuJoint block provides a way to adapt the location and orientation of a part of an object.
      |
      | For more information, please click Help.
      settings: OpenFcn=open_system([gcb '/Actuator'],'mask')
      mask Display: image(imread('Joint.png'))
  WheelL1_Audi_A8_2 : Subsystem  Tag=Actuator  Priority=0  LoadFcn=load('PrescanPoseData');load('PrescanXYZData');load('PreScanRPYData')
      mask help:
      | The VisuJoint block provides a way to adapt the location and orientation of a part of an object.
      |
      | For more information, please click Help.
      settings: OpenFcn=open_system([gcb '/Actuator'],'mask')
      mask Display: image(imread('Joint.png'))
  WheelL1_BMW_Z3_1 : Subsystem  Tag=Actuator  Priority=0  LoadFcn=load('PrescanPoseData');load('PrescanXYZData');load('PreScanRPYData')
      mask help:
      | The VisuJoint block provides a way to adapt the location and orientation of a part of an object.
      |
      | For more information, please click Help.
      settings: OpenFcn=open_system([gcb '/Actuator'],'mask')
      mask Display: image(imread('Joint.png'))
  WheelL1_BMW_Z3_2 : Subsystem  Tag=Actuator  Priority=0  LoadFcn=load('PrescanPoseData');load('PrescanXYZData');load('PreScanRPYData')
      mask help:
      | The VisuJoint block provides a way to adapt the location and orientation of a part of an object.
      |
      | For more information, please click Help.
      settings: OpenFcn=open_system([gcb '/Actuator'],'mask')
      mask Display: image(imread('Joint.png'))
  WheelL1_Citroen_C3_1 : Subsystem  Tag=Actuator  Priority=0  LoadFcn=load('PrescanPoseData');load('PrescanXYZData');load('PreScanRPYData')
      mask help:
      | The VisuJoint block provides a way to adapt the location and orientation of a part of an object.
      |
      | For more information, please click Help.
      settings: OpenFcn=open_system([gcb '/Actuator'],'mask')
      mask Display: image(imread('Joint.png'))
  WheelL1_Citroen_C3_2 : Subsystem  Tag=Actuator  Priority=0  LoadFcn=load('PrescanPoseData');load('PrescanXYZData');load('PreScanRPYData')
      mask help:
      | The VisuJoint block provides a way to adapt the location and orientation of a part of an object.
      |
      | For more information, please click Help.
      settings: OpenFcn=open_system([gcb '/Actuator'],'mask')
      mask Display: image(imread('Joint.png'))
  WheelL1_Citroen_C3_3 : Subsystem  Tag=Actuator  Priority=0  LoadFcn=load('PrescanPoseData');load('PrescanXYZData');load('PreScanRPYData')
      mask help:
      | The VisuJoint block provides a way to adapt the location and orientation of a part of an object.
      |
      | For more information, please click Help.
      settings: OpenFcn=open_system([gcb '/Actuator'],'mask')
      mask Display: image(imread('Joint.png'))
  WheelL1_Citroen_C3_4 : Subsystem  Tag=Actuator  Priority=0  LoadFcn=load('PrescanPoseData');load('PrescanXYZData');load('PreScanRPYData')
      mask help:
      | The VisuJoint block provides a way to adapt the location and orientation of a part of an object.
      |
      | For more information, please click Help.
      settings: OpenFcn=open_system([gcb '/Actuator'],'mask')
      mask Display: image(imread('Joint.png'))
  WheelL1_Fiat_Bravo_1 : Subsystem  Tag=Actuator  Priority=0  LoadFcn=load('PrescanPoseData');load('PrescanXYZData');load('PreScanRPYData')
      mask help:
      | The VisuJoint block provides a way to adapt the location and orientation of a part of an object.
      |
      | For more information, please click Help.
      settings: OpenFcn=open_system([gcb '/Actuator'],'mask')
      mask Display: image(imread('Joint.png'))
  WheelL1_Fiat_Bravo_2 : Subsystem  Tag=Actuator  Priority=0  LoadFcn=load('PrescanPoseData');load('PrescanXYZData');load('PreScanRPYData')
      mask help:
      | The VisuJoint block provides a way to adapt the location and orientation of a part of an object.
      |
      | For more information, please click Help.
      settings: OpenFcn=open_system([gcb '/Actuator'],'mask')
      mask Display: image(imread('Joint.png'))
  WheelL1_Ford_Fiesta_1 : Subsystem  Tag=Actuator  Priority=0  LoadFcn=load('PrescanPoseData');load('PrescanXYZData');load('PreScanRPYData')
      mask help:
      | The VisuJoint block provides a way to adapt the location and orientation of a part of an object.
      |
      | For more information, please click Help.
      settings: OpenFcn=open_system([gcb '/Actuator'],'mask')
      mask Display: image(imread('Joint.png'))
  WheelL1_Mazda_RX8_2 : Subsystem  Tag=Actuator  Priority=0  LoadFcn=load('PrescanPoseData');load('PrescanXYZData');load('PreScanRPYData')
      mask help:
      | The VisuJoint block provides a way to adapt the location and orientation of a part of an object.
      |
      | For more information, please click Help.
      settings: OpenFcn=open_system([gcb '/Actuator'],'mask')
      mask Display: image(imread('Joint.png'))
  WheelL1_Mazda_RX8_3 : Subsystem  Tag=Actuator  Priority=0  LoadFcn=load('PrescanPoseData');load('PrescanXYZData');load('PreScanRPYData')
      mask help:
      | The VisuJoint block provides a way to adapt the location and orientation of a part of an object.
      |
      | For more information, please click Help.
      settings: OpenFcn=open_system([gcb '/Actuator'],'mask')
      mask Display: image(imread('Joint.png'))
  WheelL1_Toyota_Previa_2 : Subsystem  Tag=Actuator  Priority=0  LoadFcn=load('PrescanPoseData');load('PrescanXYZData');load('PreScanRPYData')
      mask help:
      | The VisuJoint block provides a way to adapt the location and orientation of a part of an object.
      |
      | For more information, please click Help.
      settings: OpenFcn=open_system([gcb '/Actuator'],'mask')
      mask Display: image(imread('Joint.png'))
  WheelL1_Toyota_Yaris_1 : Subsystem  Tag=Actuator  Priority=0  LoadFcn=load('PrescanPoseData');load('PrescanXYZData');load('PreScanRPYData')
      mask help:
      | The VisuJoint block provides a way to adapt the location and orientation of a part of an object.
      |
      | For more information, please click Help.
      settings: OpenFcn=open_system([gcb '/Actuator'],'mask')
      mask Display: image(imread('Joint.png'))
  WheelR0_Actros_2541_2 : Subsystem  Tag=Actuator  Priority=0  LoadFcn=load('PrescanPoseData');load('PrescanXYZData');load('PreScanRPYData')
      mask help:
      | The VisuJoint block provides a way to adapt the location and orientation of a part of an object.
      |
      | For more information, please click Help.
      settings: OpenFcn=open_system([gcb '/Actuator'],'mask')
      mask Display: image(imread('Joint.png'))
  WheelR0_Audi_A8_1 : Subsystem  Tag=Actuator  Priority=0  LoadFcn=load('PrescanPoseData');load('PrescanXYZData');load('PreScanRPYData')
      mask help:
      | The VisuJoint block provides a way to adapt the location and orientation of a part of an object.
      |
      | For more information, please click Help.
      settings: OpenFcn=open_system([gcb '/Actuator'],'mask')
      mask Display: image(imread('Joint.png'))
  WheelR0_Audi_A8_2 : Subsystem  Tag=Actuator  Priority=0  LoadFcn=load('PrescanPoseData');load('PrescanXYZData');load('PreScanRPYData')
      mask help:
      | The VisuJoint block provides a way to adapt the location and orientation of a part of an object.
      |
      | For more information, please click Help.
      settings: OpenFcn=open_system([gcb '/Actuator'],'mask')
      mask Display: image(imread('Joint.png'))
  WheelR0_BMW_Z3_1 : Subsystem  Tag=Actuator  Priority=0  LoadFcn=load('PrescanPoseData');load('PrescanXYZData');load('PreScanRPYData')
      mask help:
      | The VisuJoint block provides a way to adapt the location and orientation of a part of an object.
      |
      | For more information, please click Help.
      settings: OpenFcn=open_system([gcb '/Actuator'],'mask')
      mask Display: image(imread('Joint.png'))
  WheelR0_BMW_Z3_2 : Subsystem  Tag=Actuator  Priority=0  LoadFcn=load('PrescanPoseData');load('PrescanXYZData');load('PreScanRPYData')
      mask help:
      | The VisuJoint block provides a way to adapt the location and orientation of a part of an object.
      |
      | For more information, please click Help.
      settings: OpenFcn=open_system([gcb '/Actuator'],'mask')
      mask Display: image(imread('Joint.png'))
  WheelR0_Citroen_C3_1 : Subsystem  Tag=Actuator  Priority=0  LoadFcn=load('PrescanPoseData');load('PrescanXYZData');load('PreScanRPYData')
      mask help:
      | The VisuJoint block provides a way to adapt the location and orientation of a part of an object.
      |
      | For more information, please click Help.
      settings: OpenFcn=open_system([gcb '/Actuator'],'mask')
      mask Display: image(imread('Joint.png'))
  WheelR0_Citroen_C3_2 : Subsystem  Tag=Actuator  Priority=0  LoadFcn=load('PrescanPoseData');load('PrescanXYZData');load('PreScanRPYData')
      mask help:
      | The VisuJoint block provides a way to adapt the location and orientation of a part of an object.
      |
      | For more information, please click Help.
      settings: OpenFcn=open_system([gcb '/Actuator'],'mask')
      mask Display: image(imread('Joint.png'))
  WheelR0_Citroen_C3_3 : Subsystem  Tag=Actuator  Priority=0  LoadFcn=load('PrescanPoseData');load('PrescanXYZData');load('PreScanRPYData')
      mask help:
      | The VisuJoint block provides a way to adapt the location and orientation of a part of an object.
      |
      | For more information, please click Help.
      settings: OpenFcn=open_system([gcb '/Actuator'],'mask')
      mask Display: image(imread('Joint.png'))
  WheelR0_Citroen_C3_4 : Subsystem  Tag=Actuator  Priority=0  LoadFcn=load('PrescanPoseData');load('PrescanXYZData');load('PreScanRPYData')
      mask help:
      | The VisuJoint block provides a way to adapt the location and orientation of a part of an object.
      |
      | For more information, please click Help.
      settings: OpenFcn=open_system([gcb '/Actuator'],'mask')
      mask Display: image(imread('Joint.png'))
  WheelR0_Fiat_Bravo_1 : Subsystem  Tag=Actuator  Priority=0  LoadFcn=load('PrescanPoseData');load('PrescanXYZData');load('PreScanRPYData')
      mask help:
      | The VisuJoint block provides a way to adapt the location and orientation of a part of an object.
      |
      | For more information, please click Help.
      settings: OpenFcn=open_system([gcb '/Actuator'],'mask')
      mask Display: image(imread('Joint.png'))
  WheelR0_Fiat_Bravo_2 : Subsystem  Tag=Actuator  Priority=0  LoadFcn=load('PrescanPoseData');load('PrescanXYZData');load('PreScanRPYData')
      mask help:
      | The VisuJoint block provides a way to adapt the location and orientation of a part of an object.
      |
      | For more information, please click Help.
      settings: OpenFcn=open_system([gcb '/Actuator'],'mask')
      mask Display: image(imread('Joint.png'))
  WheelR0_Ford_Fiesta_1 : Subsystem  Tag=Actuator  Priority=0  LoadFcn=load('PrescanPoseData');load('PrescanXYZData');load('PreScanRPYData')
      mask help:
      | The VisuJoint block provides a way to adapt the location and orientation of a part of an object.
      |
      | For more information, please click Help.
      settings: OpenFcn=open_system([gcb '/Actuator'],'mask')
      mask Display: image(imread('Joint.png'))
  WheelR0_Mazda_RX8_2 : Subsystem  Tag=Actuator  Priority=0  LoadFcn=load('PrescanPoseData');load('PrescanXYZData');load('PreScanRPYData')
      mask help:
      | The VisuJoint block provides a way to adapt the location and orientation of a part of an object.
      |
      | For more information, please click Help.
      settings: OpenFcn=open_system([gcb '/Actuator'],'mask')
      mask Display: image(imread('Joint.png'))
  WheelR0_Mazda_RX8_3 : Subsystem  Tag=Actuator  Priority=0  LoadFcn=load('PrescanPoseData');load('PrescanXYZData');load('PreScanRPYData')
      mask help:
      | The VisuJoint block provides a way to adapt the location and orientation of a part of an object.
      |
      | For more information, please click Help.
      settings: OpenFcn=open_system([gcb '/Actuator'],'mask')
      mask Display: image(imread('Joint.png'))
  WheelR0_Toyota_Previa_2 : Subsystem  Tag=Actuator  Priority=0  LoadFcn=load('PrescanPoseData');load('PrescanXYZData');load('PreScanRPYData')
      mask help:
      | The VisuJoint block provides a way to adapt the location and orientation of a part of an object.
      |
      | For more information, please click Help.
      settings: OpenFcn=open_system([gcb '/Actuator'],'mask')
      mask Display: image(imread('Joint.png'))
  WheelR0_Toyota_Yaris_1 : Subsystem  Tag=Actuator  Priority=0  LoadFcn=load('PrescanPoseData');load('PrescanXYZData');load('PreScanRPYData')
      mask help:
      | The VisuJoint block provides a way to adapt the location and orientation of a part of an object.
      |
      | For more information, please click Help.
      settings: OpenFcn=open_system([gcb '/Actuator'],'mask')
      mask Display: image(imread('Joint.png'))
  WheelR1_Actros_2541_2 : Subsystem  Tag=Actuator  Priority=0  LoadFcn=load('PrescanPoseData');load('PrescanXYZData');load('PreScanRPYData')
      mask help:
      | The VisuJoint block provides a way to adapt the location and orientation of a part of an object.
      |
      | For more information, please click Help.
      settings: OpenFcn=open_system([gcb '/Actuator'],'mask')
      mask Display: image(imread('Joint.png'))
  WheelR1_Audi_A8_1 : Subsystem  Tag=Actuator  Priority=0  LoadFcn=load('PrescanPoseData');load('PrescanXYZData');load('PreScanRPYData')
      mask help:
      | The VisuJoint block provides a way to adapt the location and orientation of a part of an object.
      |
      | For more information, please click Help.
      settings: OpenFcn=open_system([gcb '/Actuator'],'mask')
      mask Display: image(imread('Joint.png'))
  WheelR1_Audi_A8_2 : Subsystem  Tag=Actuator  Priority=0  LoadFcn=load('PrescanPoseData');load('PrescanXYZData');load('PreScanRPYData')
      mask help:
      | The VisuJoint block provides a way to adapt the location and orientation of a part of an object.
      |
      | For more information, please click Help.
      settings: OpenFcn=open_system([gcb '/Actuator'],'mask')
      mask Display: image(imread('Joint.png'))
  WheelR1_BMW_Z3_1 : Subsystem  Tag=Actuator  Priority=0  LoadFcn=load('PrescanPoseData');load('PrescanXYZData');load('PreScanRPYData')
      mask help:
      | The VisuJoint block provides a way to adapt the location and orientation of a part of an object.
      |
      | For more information, please click Help.
      settings: OpenFcn=open_system([gcb '/Actuator'],'mask')
      mask Display: image(imread('Joint.png'))
  WheelR1_BMW_Z3_2 : Subsystem  Tag=Actuator  Priority=0  LoadFcn=load('PrescanPoseData');load('PrescanXYZData');load('PreScanRPYData')
      mask help:
      | The VisuJoint block provides a way to adapt the location and orientation of a part of an object.
      |
      | For more information, please click Help.
      settings: OpenFcn=open_system([gcb '/Actuator'],'mask')
      mask Display: image(imread('Joint.png'))
  WheelR1_Citroen_C3_1 : Subsystem  Tag=Actuator  Priority=0  LoadFcn=load('PrescanPoseData');load('PrescanXYZData');load('PreScanRPYData')
      mask help:
      | The VisuJoint block provides a way to adapt the location and orientation of a part of an object.
      |
      | For more information, please click Help.
      settings: OpenFcn=open_system([gcb '/Actuator'],'mask')
      mask Display: image(imread('Joint.png'))
  WheelR1_Citroen_C3_2 : Subsystem  Tag=Actuator  Priority=0  LoadFcn=load('PrescanPoseData');load('PrescanXYZData');load('PreScanRPYData')
      mask help:
      | The VisuJoint block provides a way to adapt the location and orientation of a part of an object.
      |
      | For more information, please click Help.
      settings: OpenFcn=open_system([gcb '/Actuator'],'mask')
      mask Display: image(imread('Joint.png'))
  WheelR1_Citroen_C3_3 : Subsystem  Tag=Actuator  Priority=0  LoadFcn=load('PrescanPoseData');load('PrescanXYZData');load('PreScanRPYData')
      mask help:
      | The VisuJoint block provides a way to adapt the location and orientation of a part of an object.
      |
      | For more information, please click Help.
      settings: OpenFcn=open_system([gcb '/Actuator'],'mask')
      mask Display: image(imread('Joint.png'))
  WheelR1_Citroen_C3_4 : Subsystem  Tag=Actuator  Priority=0  LoadFcn=load('PrescanPoseData');load('PrescanXYZData');load('PreScanRPYData')
      mask help:
      | The VisuJoint block provides a way to adapt the location and orientation of a part of an object.
      |
      | For more information, please click Help.
      settings: OpenFcn=open_system([gcb '/Actuator'],'mask')
      mask Display: image(imread('Joint.png'))
  WheelR1_Fiat_Bravo_1 : Subsystem  Tag=Actuator  Priority=0  LoadFcn=load('PrescanPoseData');load('PrescanXYZData');load('PreScanRPYData')
      mask help:
      | The VisuJoint block provides a way to adapt the location and orientation of a part of an object.
      |
      | For more information, please click Help.
      settings: OpenFcn=open_system([gcb '/Actuator'],'mask')
      mask Display: image(imread('Joint.png'))
  WheelR1_Fiat_Bravo_2 : Subsystem  Tag=Actuator  Priority=0  LoadFcn=load('PrescanPoseData');load('PrescanXYZData');load('PreScanRPYData')
      mask help:
      | The VisuJoint block provides a way to adapt the location and orientation of a part of an object.
      |
      | For more information, please click Help.
      settings: OpenFcn=open_system([gcb '/Actuator'],'mask')
      mask Display: image(imread('Joint.png'))
  WheelR1_Ford_Fiesta_1 : Subsystem  Tag=Actuator  Priority=0  LoadFcn=load('PrescanPoseData');load('PrescanXYZData');load('PreScanRPYData')
      mask help:
      | The VisuJoint block provides a way to adapt the location and orientation of a part of an object.
      |
      | For more information, please click Help.
      settings: OpenFcn=open_system([gcb '/Actuator'],'mask')
      mask Display: image(imread('Joint.png'))
  WheelR1_Mazda_RX8_2 : Subsystem  Tag=Actuator  Priority=0  LoadFcn=load('PrescanPoseData');load('PrescanXYZData');load('PreScanRPYData')
      mask help:
      | The VisuJoint block provides a way to adapt the location and orientation of a part of an object.
      |
      | For more information, please click Help.
      settings: OpenFcn=open_system([gcb '/Actuator'],'mask')
      mask Display: image(imread('Joint.png'))
  WheelR1_Mazda_RX8_3 : Subsystem  Tag=Actuator  Priority=0  LoadFcn=load('PrescanPoseData');load('PrescanXYZData');load('PreScanRPYData')
      mask help:
      | The VisuJoint block provides a way to adapt the location and orientation of a part of an object.
      |
      | For more information, please click Help.
      settings: OpenFcn=open_system([gcb '/Actuator'],'mask')
      mask Display: image(imread('Joint.png'))
  WheelR1_Toyota_Previa_2 : Subsystem  Tag=Actuator  Priority=0  LoadFcn=load('PrescanPoseData');load('PrescanXYZData');load('PreScanRPYData')
      mask help:
      | The VisuJoint block provides a way to adapt the location and orientation of a part of an object.
      |
      | For more information, please click Help.
      settings: OpenFcn=open_system([gcb '/Actuator'],'mask')
      mask Display: image(imread('Joint.png'))
  WheelR1_Toyota_Yaris_1 : Subsystem  Tag=Actuator  Priority=0  LoadFcn=load('PrescanPoseData');load('PrescanXYZData');load('PreScanRPYData')
      mask help:
      | The VisuJoint block provides a way to adapt the location and orientation of a part of an object.
      |
      | For more information, please click Help.
      settings: OpenFcn=open_system([gcb '/Actuator'],'mask')
      mask Display: image(imread('Joint.png'))
  wires:
  Audi_A8_1/1(STATE_Audi_A8_1_bus) -> STATE_Audi_A8_1_bus/1(STATE_Audi_A8_1_bus)
  SELF_Audi_A8_1/1(SELF_Audi_A8_1) -> Audi_A8_1/1(SELF_Audi_A8_1)
  CameraSensor_1/1(CameraSensor_1) -> Audi_A8_1/2(CameraSensor_1)
  Audi_A8_1/2(WheelL0_Audi_A8_1) -> WheelL0_Audi_A8_1/1(WheelL0_Audi_A8_1)
  Audi_A8_1/3(WheelL1_Audi_A8_1) -> WheelL1_Audi_A8_1/1(WheelL1_Audi_A8_1)
  Audi_A8_1/4(WheelR0_Audi_A8_1) -> WheelR0_Audi_A8_1/1(WheelR0_Audi_A8_1)
  Audi_A8_1/5(WheelR1_Audi_A8_1) -> WheelR1_Audi_A8_1/1(WheelR1_Audi_A8_1)
  Audi_A8_1/6(SteeringWheel_pivot_Audi_A8_1) -> SteeringWheel_pivot_Audi_A8_1/1(SteeringWheel_pivot_Audi_A8_1)
  Audi_A8_1/7(SteeringColumn_pivot_Audi_A8_1) -> SteeringColumn_pivot_Audi_A8_1/1(SteeringColumn_pivot_Audi_A8_1)
  Audi_A8_1/8(Audi_A8_1_Brake_light_left) -> Audi_A8_1_Brake_light_left/1(Audi_A8_1_Brake_light_left)
  Audi_A8_1/9(Audi_A8_1_Brake_light_right) -> Audi_A8_1_Brake_light_right/1(Audi_A8_1_Brake_light_right)
  Audi_A8_1/10(Audi_A8_1_Indicator_front_left) -> Audi_A8_1_Indicator_front_left/1(Audi_A8_1_Indicator_front_left)
  Audi_A8_1/11(Audi_A8_1_Indicator_rear_left) -> Audi_A8_1_Indicator_rear_left/1(Audi_A8_1_Indicator_rear_left)
  Audi_A8_1/12(Audi_A8_1_Indicator_front_right) -> Audi_A8_1_Indicator_front_right/1(Audi_A8_1_Indicator_front_right)
  Audi_A8_1/13(Audi_A8_1_Indicator_rear_right) -> Audi_A8_1_Indicator_rear_right/1(Audi_A8_1_Indicator_rear_right)
  Sphere_1/1(STATE_Sphere_1_bus) -> STATE_Sphere_1_bus/1(STATE_Sphere_1_bus)
  SELF_Sphere_1/1(SELF_Sphere_1) -> Sphere_1/1(SELF_Sphere_1)
  Nissan_Cabstar_1/1(STATE_Nissan_Cabstar_1_bus) -> STATE_Nissan_Cabstar_1_bus/1(STATE_Nissan_Cabstar_1_bus)
  SELF_Nissan_Cabstar_1/1(SELF_Nissan_Cabstar_1) -> Nissan_Cabstar_1/1(SELF_Nissan_Cabstar_1)
  Nissan_Cabstar_1/2(VISUColorRegion_Exterior_Nissan_Cabstar_1) -> VISUColorRegion_Exterior_Nissan_Cabstar_1/1(VISUColorRegion_Exterior_Nissan_Cabstar_1)
  Actros_1860_1/1(STATE_Actros_1860_1_bus) -> STATE_Actros_1860_1_bus/1(STATE_Actros_1860_1_bus)
  SELF_Actros_1860_1/1(SELF_Actros_1860_1) -> Actros_1860_1/1(SELF_Actros_1860_1)
  ContainerTrailer_DoubleAxle_1/1(STATE_ContainerTrailer_DoubleAxle_1_bus) -> STATE_ContainerTrailer_DoubleAxle_1_bus/1(STATE_ContainerTrailer_DoubleAxle_1_bus)
  SELF_ContainerTrailer_DoubleAxle_1/1(SELF_ContainerTrailer_DoubleAxle_1) -> ContainerTrailer_DoubleAxle_1/1(SELF_ContainerTrailer_DoubleAxle_1)
  Actros_1860_2/1(STATE_Actros_1860_2_bus) -> STATE_Actros_1860_2_bus/1(STATE_Actros_1860_2_bus)
  SELF_Actros_1860_2/1(SELF_Actros_1860_2) -> Actros_1860_2/1(SELF_Actros_1860_2)
  ContainerTrailer_DoubleAxle_2/1(STATE_ContainerTrailer_DoubleAxle_2_bus) -> STATE_ContainerTrailer_DoubleAxle_2_bus/1(STATE_ContainerTrailer_DoubleAxle_2_bus)
  SELF_ContainerTrailer_DoubleAxle_2/1(SELF_ContainerTrailer_DoubleAxle_2) -> ContainerTrailer_DoubleAxle_2/1(SELF_ContainerTrailer_DoubleAxle_2)
  Actros_2541_1/1(STATE_Actros_2541_1_bus) -> STATE_Actros_2541_1_bus/1(STATE_Actros_2541_1_bus)
  SELF_Actros_2541_1/1(SELF_Actros_2541_1) -> Actros_2541_1/1(SELF_Actros_2541_1)
  Toyota_Previa_1/1(STATE_Toyota_Previa_1_bus) -> STATE_Toyota_Previa_1_bus/1(STATE_Toyota_Previa_1_bus)
  SELF_Toyota_Previa_1/1(SELF_Toyota_Previa_1) -> Toyota_Previa_1/1(SELF_Toyota_Previa_1)
  Toyota_Previa_1/2(VISUColorRegion_Exterior_Toyota_Previa_1) -> VISUColorRegion_Exterior_Toyota_Previa_1/1(VISUColorRegion_Exterior_Toyota_Previa_1)
  Mazda_RX8_1/1(STATE_Mazda_RX8_1_bus) -> STATE_Mazda_RX8_1_bus/1(STATE_Mazda_RX8_1_bus)
  SELF_Mazda_RX8_1/1(SELF_Mazda_RX8_1) -> Mazda_RX8_1/1(SELF_Mazda_RX8_1)
  Mazda_RX8_1/2(VISUColorRegion_Exterior_Mazda_RX8_1) -> VISUColorRegion_Exterior_Mazda_RX8_1/1(VISUColorRegion_Exterior_Mazda_RX8_1)
  Mazda_RX8_2/1(STATE_Mazda_RX8_2_bus) -> STATE_Mazda_RX8_2_bus/1(STATE_Mazda_RX8_2_bus)
  SELF_Mazda_RX8_2/1(SELF_Mazda_RX8_2) -> Mazda_RX8_2/1(SELF_Mazda_RX8_2)
  Mazda_RX8_2/2(WheelL0_Mazda_RX8_2) -> WheelL0_Mazda_RX8_2/1(WheelL0_Mazda_RX8_2)
  Mazda_RX8_2/3(WheelL1_Mazda_RX8_2) -> WheelL1_Mazda_RX8_2/1(WheelL1_Mazda_RX8_2)
  Mazda_RX8_2/4(WheelR0_Mazda_RX8_2) -> WheelR0_Mazda_RX8_2/1(WheelR0_Mazda_RX8_2)
  Mazda_RX8_2/5(WheelR1_Mazda_RX8_2) -> WheelR1_Mazda_RX8_2/1(WheelR1_Mazda_RX8_2)
  Mazda_RX8_2/6(VISUColorRegion_Exterior_Mazda_RX8_2) -> VISUColorRegion_Exterior_Mazda_RX8_2/1(VISUColorRegion_Exterior_Mazda_RX8_2)
  Ford_Fiesta_1/1(STATE_Ford_Fiesta_1_bus) -> STATE_Ford_Fiesta_1_bus/1(STATE_Ford_Fiesta_1_bus)
  SELF_Ford_Fiesta_1/1(SELF_Ford_Fiesta_1) -> Ford_Fiesta_1/1(SELF_Ford_Fiesta_1)
  Ford_Fiesta_1/2(WheelL0_Ford_Fiesta_1) -> WheelL0_Ford_Fiesta_1/1(WheelL0_Ford_Fiesta_1)
  Ford_Fiesta_1/3(WheelL1_Ford_Fiesta_1) -> WheelL1_Ford_Fiesta_1/1(WheelL1_Ford_Fiesta_1)
  Ford_Fiesta_1/4(WheelR0_Ford_Fiesta_1) -> WheelR0_Ford_Fiesta_1/1(WheelR0_Ford_Fiesta_1)
  Ford_Fiesta_1/5(WheelR1_Ford_Fiesta_1) -> WheelR1_Ford_Fiesta_1/1(WheelR1_Ford_Fiesta_1)
  Ford_Fiesta_1/6(VISUColorRegion_Exterior_Ford_Fiesta_1) -> VISUColorRegion_Exterior_Ford_Fiesta_1/1(VISUColorRegion_Exterior_Ford_Fiesta_1)
  BMW_Z3_1/1(STATE_BMW_Z3_1_bus) -> STATE_BMW_Z3_1_bus/1(STATE_BMW_Z3_1_bus)
  SELF_BMW_Z3_1/1(SELF_BMW_Z3_1) -> BMW_Z3_1/1(SELF_BMW_Z3_1)
  BMW_Z3_1/2(WheelL0_BMW_Z3_1) -> WheelL0_BMW_Z3_1/1(WheelL0_BMW_Z3_1)
  BMW_Z3_1/3(WheelL1_BMW_Z3_1) -> WheelL1_BMW_Z3_1/1(WheelL1_BMW_Z3_1)
  BMW_Z3_1/4(WheelR0_BMW_Z3_1) -> WheelR0_BMW_Z3_1/1(WheelR0_BMW_Z3_1)
  BMW_Z3_1/5(WheelR1_BMW_Z3_1) -> WheelR1_BMW_Z3_1/1(WheelR1_BMW_Z3_1)
  BMW_Z3_1/6(VISUColorRegion_Exterior_BMW_Z3_1) -> VISUColorRegion_Exterior_BMW_Z3_1/1(VISUColorRegion_Exterior_BMW_Z3_1)
  Audi_A8_2/1(STATE_Audi_A8_2_bus) -> STATE_Audi_A8_2_bus/1(STATE_Audi_A8_2_bus)
  SELF_Audi_A8_2/1(SELF_Audi_A8_2) -> Audi_A8_2/1(SELF_Audi_A8_2)
  Audi_A8_2/2(WheelL0_Audi_A8_2) -> WheelL0_Audi_A8_2/1(WheelL0_Audi_A8_2)
  Audi_A8_2/3(WheelL1_Audi_A8_2) -> WheelL1_Audi_A8_2/1(WheelL1_Audi_A8_2)
  Audi_A8_2/4(WheelR0_Audi_A8_2) -> WheelR0_Audi_A8_2/1(WheelR0_Audi_A8_2)
  Audi_A8_2/5(WheelR1_Audi_A8_2) -> WheelR1_Audi_A8_2/1(WheelR1_Audi_A8_2)
  Audi_A8_2/6(VISUColorRegion_Exterior_Audi_A8_2) -> VISUColorRegion_Exterior_Audi_A8_2/1(VISUColorRegion_Exterior_Audi_A8_2)
  Citroen_C3_1/1(STATE_Citroen_C3_1_bus) -> STATE_Citroen_C3_1_bus/1(STATE_Citroen_C3_1_bus)
  SELF_Citroen_C3_1/1(SELF_Citroen_C3_1) -> Citroen_C3_1/1(SELF_Citroen_C3_1)
  Citroen_C3_1/2(WheelL0_Citroen_C3_1) -> WheelL0_Citroen_C3_1/1(WheelL0_Citroen_C3_1)
  Citroen_C3_1/3(WheelL1_Citroen_C3_1) -> WheelL1_Citroen_C3_1/1(WheelL1_Citroen_C3_1)
  Citroen_C3_1/4(WheelR0_Citroen_C3_1) -> WheelR0_Citroen_C3_1/1(WheelR0_Citroen_C3_1)
  Citroen_C3_1/5(WheelR1_Citroen_C3_1) -> WheelR1_Citroen_C3_1/1(WheelR1_Citroen_C3_1)
  Citroen_C3_1/6(VISUColorRegion_Exterior_Citroen_C3_1) -> VISUColorRegion_Exterior_Citroen_C3_1/1(VISUColorRegion_Exterior_Citroen_C3_1)
  Citroen_C3_2/1(STATE_Citroen_C3_2_bus) -> STATE_Citroen_C3_2_bus/1(STATE_Citroen_C3_2_bus)
  SELF_Citroen_C3_2/1(SELF_Citroen_C3_2) -> Citroen_C3_2/1(SELF_Citroen_C3_2)
  Citroen_C3_2/2(WheelL0_Citroen_C3_2) -> WheelL0_Citroen_C3_2/1(WheelL0_Citroen_C3_2)
  Citroen_C3_2/3(WheelL1_Citroen_C3_2) -> WheelL1_Citroen_C3_2/1(WheelL1_Citroen_C3_2)
  Citroen_C3_2/4(WheelR0_Citroen_C3_2) -> WheelR0_Citroen_C3_2/1(WheelR0_Citroen_C3_2)
  Citroen_C3_2/5(WheelR1_Citroen_C3_2) -> WheelR1_Citroen_C3_2/1(WheelR1_Citroen_C3_2)
  Citroen_C3_2/6(VISUColorRegion_Exterior_Citroen_C3_2) -> VISUColorRegion_Exterior_Citroen_C3_2/1(VISUColorRegion_Exterior_Citroen_C3_2)
  Toyota_Yaris_1/1(STATE_Toyota_Yaris_1_bus) -> STATE_Toyota_Yaris_1_bus/1(STATE_Toyota_Yaris_1_bus)
  SELF_Toyota_Yaris_1/1(SELF_Toyota_Yaris_1) -> Toyota_Yaris_1/1(SELF_Toyota_Yaris_1)
  Toyota_Yaris_1/2(WheelL0_Toyota_Yaris_1) -> WheelL0_Toyota_Yaris_1/1(WheelL0_Toyota_Yaris_1)
  Toyota_Yaris_1/3(WheelL1_Toyota_Yaris_1) -> WheelL1_Toyota_Yaris_1/1(WheelL1_Toyota_Yaris_1)
  Toyota_Yaris_1/4(WheelR0_Toyota_Yaris_1) -> WheelR0_Toyota_Yaris_1/1(WheelR0_Toyota_Yaris_1)
  Toyota_Yaris_1/5(WheelR1_Toyota_Yaris_1) -> WheelR1_Toyota_Yaris_1/1(WheelR1_Toyota_Yaris_1)
  Toyota_Yaris_1/6(VISUColorRegion_Exterior_Toyota_Yaris_1) -> VISUColorRegion_Exterior_Toyota_Yaris_1/1(VISUColorRegion_Exterior_Toyota_Yaris_1)
  Fiat_Bravo_1/1(STATE_Fiat_Bravo_1_bus) -> STATE_Fiat_Bravo_1_bus/1(STATE_Fiat_Bravo_1_bus)
  SELF_Fiat_Bravo_1/1(SELF_Fiat_Bravo_1) -> Fiat_Bravo_1/1(SELF_Fiat_Bravo_1)
  Fiat_Bravo_1/2(WheelL0_Fiat_Bravo_1) -> WheelL0_Fiat_Bravo_1/1(WheelL0_Fiat_Bravo_1)
  Fiat_Bravo_1/3(WheelL1_Fiat_Bravo_1) -> WheelL1_Fiat_Bravo_1/1(WheelL1_Fiat_Bravo_1)
  Fiat_Bravo_1/4(WheelR0_Fiat_Bravo_1) -> WheelR0_Fiat_Bravo_1/1(WheelR0_Fiat_Bravo_1)
  Fiat_Bravo_1/5(WheelR1_Fiat_Bravo_1) -> WheelR1_Fiat_Bravo_1/1(WheelR1_Fiat_Bravo_1)
  Fiat_Bravo_1/6(VISUColorRegion_Exterior_Fiat_Bravo_1) -> VISUColorRegion_Exterior_Fiat_Bravo_1/1(VISUColorRegion_Exterior_Fiat_Bravo_1)
  Citroen_C3_3/1(STATE_Citroen_C3_3_bus) -> STATE_Citroen_C3_3_bus/1(STATE_Citroen_C3_3_bus)
  SELF_Citroen_C3_3/1(SELF_Citroen_C3_3) -> Citroen_C3_3/1(SELF_Citroen_C3_3)
  Citroen_C3_3/2(WheelL0_Citroen_C3_3) -> WheelL0_Citroen_C3_3/1(WheelL0_Citroen_C3_3)
  Citroen_C3_3/3(WheelL1_Citroen_C3_3) -> WheelL1_Citroen_C3_3/1(WheelL1_Citroen_C3_3)
  Citroen_C3_3/4(WheelR0_Citroen_C3_3) -> WheelR0_Citroen_C3_3/1(WheelR0_Citroen_C3_3)
  Citroen_C3_3/5(WheelR1_Citroen_C3_3) -> WheelR1_Citroen_C3_3/1(WheelR1_Citroen_C3_3)
  Citroen_C3_3/6(VISUColorRegion_Exterior_Citroen_C3_3) -> VISUColorRegion_Exterior_Citroen_C3_3/1(VISUColorRegion_Exterior_Citroen_C3_3)
  Toyota_Previa_2/1(STATE_Toyota_Previa_2_bus) -> STATE_Toyota_Previa_2_bus/1(STATE_Toyota_Previa_2_bus)
  SELF_Toyota_Previa_2/1(SELF_Toyota_Previa_2) -> Toyota_Previa_2/1(SELF_Toyota_Previa_2)
  Toyota_Previa_2/2(WheelL0_Toyota_Previa_2) -> WheelL0_Toyota_Previa_2/1(WheelL0_Toyota_Previa_2)
  Toyota_Previa_2/3(WheelL1_Toyota_Previa_2) -> WheelL1_Toyota_Previa_2/1(WheelL1_Toyota_Previa_2)
  Toyota_Previa_2/4(WheelR0_Toyota_Previa_2) -> WheelR0_Toyota_Previa_2/1(WheelR0_Toyota_Previa_2)
  Toyota_Previa_2/5(WheelR1_Toyota_Previa_2) -> WheelR1_Toyota_Previa_2/1(WheelR1_Toyota_Previa_2)
  Toyota_Previa_2/6(VISUColorRegion_Exterior_Toyota_Previa_2) -> VISUColorRegion_Exterior_Toyota_Previa_2/1(VISUColorRegion_Exterior_Toyota_Previa_2)
  Mazda_RX8_3/1(STATE_Mazda_RX8_3_bus) -> STATE_Mazda_RX8_3_bus/1(STATE_Mazda_RX8_3_bus)
  SELF_Mazda_RX8_3/1(SELF_Mazda_RX8_3) -> Mazda_RX8_3/1(SELF_Mazda_RX8_3)
  Mazda_RX8_3/2(WheelL0_Mazda_RX8_3) -> WheelL0_Mazda_RX8_3/1(WheelL0_Mazda_RX8_3)
  Mazda_RX8_3/3(WheelL1_Mazda_RX8_3) -> WheelL1_Mazda_RX8_3/1(WheelL1_Mazda_RX8_3)
  Mazda_RX8_3/4(WheelR0_Mazda_RX8_3) -> WheelR0_Mazda_RX8_3/1(WheelR0_Mazda_RX8_3)
  Mazda_RX8_3/5(WheelR1_Mazda_RX8_3) -> WheelR1_Mazda_RX8_3/1(WheelR1_Mazda_RX8_3)
  Mazda_RX8_3/6(VISUColorRegion_Exterior_Mazda_RX8_3) -> VISUColorRegion_Exterior_Mazda_RX8_3/1(VISUColorRegion_Exterior_Mazda_RX8_3)
  Fiat_Bravo_2/1(STATE_Fiat_Bravo_2_bus) -> STATE_Fiat_Bravo_2_bus/1(STATE_Fiat_Bravo_2_bus)
  SELF_Fiat_Bravo_2/1(SELF_Fiat_Bravo_2) -> Fiat_Bravo_2/1(SELF_Fiat_Bravo_2)
  Fiat_Bravo_2/2(WheelL0_Fiat_Bravo_2) -> WheelL0_Fiat_Bravo_2/1(WheelL0_Fiat_Bravo_2)
  Fiat_Bravo_2/3(WheelL1_Fiat_Bravo_2) -> WheelL1_Fiat_Bravo_2/1(WheelL1_Fiat_Bravo_2)
  Fiat_Bravo_2/4(WheelR0_Fiat_Bravo_2) -> WheelR0_Fiat_Bravo_2/1(WheelR0_Fiat_Bravo_2)
  Fiat_Bravo_2/5(WheelR1_Fiat_Bravo_2) -> WheelR1_Fiat_Bravo_2/1(WheelR1_Fiat_Bravo_2)
  BMW_Z3_2/1(STATE_BMW_Z3_2_bus) -> STATE_BMW_Z3_2_bus/1(STATE_BMW_Z3_2_bus)
  SELF_BMW_Z3_2/1(SELF_BMW_Z3_2) -> BMW_Z3_2/1(SELF_BMW_Z3_2)
  BMW_Z3_2/2(WheelL0_BMW_Z3_2) -> WheelL0_BMW_Z3_2/1(WheelL0_BMW_Z3_2)
  BMW_Z3_2/3(WheelL1_BMW_Z3_2) -> WheelL1_BMW_Z3_2/1(WheelL1_BMW_Z3_2)
  BMW_Z3_2/4(WheelR0_BMW_Z3_2) -> WheelR0_BMW_Z3_2/1(WheelR0_BMW_Z3_2)
  BMW_Z3_2/5(WheelR1_BMW_Z3_2) -> WheelR1_BMW_Z3_2/1(WheelR1_BMW_Z3_2)
  BMW_Z3_2/6(VISUColorRegion_Exterior_BMW_Z3_2) -> VISUColorRegion_Exterior_BMW_Z3_2/1(VISUColorRegion_Exterior_BMW_Z3_2)
  Citroen_C3_4/1(STATE_Citroen_C3_4_bus) -> STATE_Citroen_C3_4_bus/1(STATE_Citroen_C3_4_bus)
  SELF_Citroen_C3_4/1(SELF_Citroen_C3_4) -> Citroen_C3_4/1(SELF_Citroen_C3_4)
  Citroen_C3_4/2(WheelL0_Citroen_C3_4) -> WheelL0_Citroen_C3_4/1(WheelL0_Citroen_C3_4)
  Citroen_C3_4/3(WheelL1_Citroen_C3_4) -> WheelL1_Citroen_C3_4/1(WheelL1_Citroen_C3_4)
  Citroen_C3_4/4(WheelR0_Citroen_C3_4) -> WheelR0_Citroen_C3_4/1(WheelR0_Citroen_C3_4)
  Citroen_C3_4/5(WheelR1_Citroen_C3_4) -> WheelR1_Citroen_C3_4/1(WheelR1_Citroen_C3_4)
  Citroen_C3_4/6(VISUColorRegion_Exterior_Citroen_C3_4) -> VISUColorRegion_Exterior_Citroen_C3_4/1(VISUColorRegion_Exterior_Citroen_C3_4)
  Actros_2541_2/1(STATE_Actros_2541_2_bus) -> STATE_Actros_2541_2_bus/1(STATE_Actros_2541_2_bus)
  SELF_Actros_2541_2/1(SELF_Actros_2541_2) -> Actros_2541_2/1(SELF_Actros_2541_2)
  Actros_2541_2/2(WheelL0_Actros_2541_2) -> WheelL0_Actros_2541_2/1(WheelL0_Actros_2541_2)
  Actros_2541_2/3(WheelL1_Actros_2541_2) -> WheelL1_Actros_2541_2/1(WheelL1_Actros_2541_2)
  Actros_2541_2/4(WheelR0_Actros_2541_2) -> WheelR0_Actros_2541_2/1(WheelR0_Actros_2541_2)
  Actros_2541_2/5(WheelR1_Actros_2541_2) -> WheelR1_Actros_2541_2/1(WheelR1_Actros_2541_2)
  HighwayOverhang_1/1(VISUMatrixSign_HighwayOverhang_1) -> VISUMatrixSign_HighwayOverhang_1/1(VISUMatrixSign_HighwayOverhang_1)
  HighwayOverhang_1/2(VISUMatrixSignLights_HighwayOverhang_1) -> VISUMatrixSignLights_HighwayOverhang_1/1(VISUMatrixSignLights_HighwayOverhang_1)
  HighwayOverhang_2/1(VISUMatrixSign_HighwayOverhang_2) -> VISUMatrixSign_HighwayOverhang_2/1(VISUMatrixSign_HighwayOverhang_2)
  HighwayOverhang_2/2(VISUMatrixSignLights_HighwayOverhang_2) -> VISUMatrixSignLights_HighwayOverhang_2/1(VISUMatrixSignLights_HighwayOverhang_2)
  HighwayOverhang_3/1(VISUMatrixSign_HighwayOverhang_3) -> VISUMatrixSign_HighwayOverhang_3/1(VISUMatrixSign_HighwayOverhang_3)
  HighwayOverhang_3/2(VISUMatrixSignLights_HighwayOverhang_3) -> VISUMatrixSignLights_HighwayOverhang_3/1(VISUMatrixSignLights_HighwayOverhang_3)
  HighwayOverhang_4/1(VISUMatrixSign_HighwayOverhang_4) -> VISUMatrixSign_HighwayOverhang_4/1(VISUMatrixSign_HighwayOverhang_4)
  HighwayOverhang_4/2(VISUMatrixSignLights_HighwayOverhang_4) -> VISUMatrixSignLights_HighwayOverhang_4/1(VISUMatrixSignLights_HighwayOverhang_4)
  HighwayOverhang_5/1(VISUMatrixSign_HighwayOverhang_5) -> VISUMatrixSign_HighwayOverhang_5/1(VISUMatrixSign_HighwayOverhang_5)
  HighwayOverhang_5/2(VISUMatrixSignLights_HighwayOverhang_5) -> VISUMatrixSignLights_HighwayOverhang_5/1(VISUMatrixSignLights_HighwayOverhang_5)
  HighwayOverhang_6/1(VISUMatrixSign_HighwayOverhang_6) -> VISUMatrixSign_HighwayOverhang_6/1(VISUMatrixSign_HighwayOverhang_6)
  HighwayOverhang_6/2(VISUMatrixSignLights_HighwayOverhang_6) -> VISUMatrixSignLights_HighwayOverhang_6/1(VISUMatrixSignLights_HighwayOverhang_6)
  HighwayOverhang_7/1(VISUMatrixSign_HighwayOverhang_7) -> VISUMatrixSign_HighwayOverhang_7/1(VISUMatrixSign_HighwayOverhang_7)
